simulink model "VACModel"  (Simulink 8.3)
(part 6 of 18)

      |         SW_signal = evalin('base', SW_signal);
      |         if ~isvector(SW_signal)
      |             set_param(gcb, 'signalin', '');
      |             set_param([gcb '/SignalIn'], 'VariableName', '[]');
      |             warning(['Variable ' SW_signal ' must be a vector.']);
      |             clear SW_signal;
      |             return;
      |         end
      |         SW_stime = str2num(get_param(gcb, 'stime'));
      |         if isempty(SW_stime) || SW_stime < -1 || (SW_stime < 0 && SW_stime > -1)
      |             set_param(gcb, 'stime', '-1');
      |             SW_stime = -1;
      |             warning('Sample time must be a positive double or -1 for inherited value.');
      |         end
      | 
      |         if SW_stime == 0 || SW_stime == -1
      |             SW_stime = evalin('base', 'Ts_base');
      |         end
      | 
      |         SW_start = str2num(get_param(gcb, 'start'));
      |         SW_start = SW_stime * ceil(SW_start/SW_stime);
      |         signalstruct.time = SW_start:SW_stime:(SW_stime*(length(SW_signal) - 1) + SW_start);
      |         signalstruct.signals.values = SW_signal;
      | 
      | 		if strcmp(get_param(gcb, 'afterend'), 'Cyclic repetition')
      | 			SW_end = str2double(get_param(gcr, 'StopTime'));
      | 			while signalstruct.time(end) < SW_end
      | 				signalstruct.signals.values = [signalstruct.signals.values signalstruct.signals.values];
      | 				signalstruct.time = [signalstruct.time signalstruct.time+(signalstruct.time(end)-signalstruct.time(1))];
      | 			end
      | 		end
      | 
      | 		signalstruct.signals.values = signalstruct.signals.values(:);
      | 		signalstruct.time = signalstruct.time(:);
      |         %assignin('base', 'signalstruct', signalstruct)
      |         set_param([gcb '/SignalIn'], 'VariableName', 'signalstruct');
      |     end
      | 
      |     clear SW_signal;
      | 	clear SW_start;
      |     clear SW_stime;
      | 	clear SW_end;
      | elseif ~strcmpi(get_param(gcb, 'switch_mode'), 'Custom attack') && exists_block([gcb '/SignalIn']) % delete block
      |     delete_line(gcb, 'SignalIn/1', 'Multiport Switch/3');
      |     delete_block([gcb '/SignalIn']);
      |     % replace with constant value
      |     add_block(['built-in/Constant'], [gcb '/ReplaceBlock'], 'Position', [50 400 120 430]);
      |     add_line(gcb, ['ReplaceBlock/1'], 'Multiport Switch/3', 'autorouting', 'on');
      | end
      mask TypeOptions atkMode: Attack Type Controller/atkMode
      mask Callback atkMode:
      | AM_MaskEnables = get_param(gcb, 'MaskEnables');
      | switch get_param(gcb, 'atkMode');
      |     case 'No attack'
      |         AM_MaskEnables{3} = 'off';
      |         AM_MaskEnables{4} = 'off';
      |     case 'Step attack'
      |         AM_MaskEnables{3} = 'on';
      |         AM_MaskEnables{4} = 'off';
      |     otherwise
      |         AM_MaskEnables{3} = 'on';
      |         AM_MaskEnables{4} = 'on';
      | end
      | set_param(gcb, 'MaskEnables', AM_MaskEnables);
      | 
      | clear AM_MaskEnables;
      mask Callback start:
      | SS_start = get_param(gcb, 'start');
      | if strcmp(SS_start, '') % empty
      |     set_param(gcb, 'start', '0');
      |     SS_start = 0;
      | end
      | SS_start = str2num(SS_start);
      | if isempty(SS_start)
      |     set_param(gcb, 'start', '0');
      |     SS_start = 0;
      |     warning('Parameter value must be a nimeric value.');
      | end
      | 
      | % set to the subsystem
      | set_param([gcb '/Attack Type Controller'], 'start', get_param(gcb, 'start'));
      | 
      | % get correct signal parameters
      | if strcmpi(get_param(gcb, 'switch_mode'),'custom attack')
      |     if ~exists_block([gcb '/SignalIn'])
      |         clear SS_start;
      |         return
      |     end
      |     % forward signal parameters if set
      |     SS_signal = get_param(gcb, 'signalin');
      |     if strcmp(SS_signal, '[]') || strcmp(SS_signal, '') % signal not set
      |         clear SS_signal;
      |         clear SS_start;
      |         return;
      |     else    % signal set
      |         SS_signal = evalin('base', SS_signal);
      |         SS_stime = str2num(get_param(gcb, 'stime'));
      |         if isempty(SS_stime) || SS_stime < -1 || (SS_stime < 0 && SS_stime > -1)
      |             clear SS_signal;
      |             clear SS_start;
      |             set_param(gcb, 'stime', '-1');
      |             SS_stime = -1;
      |             warning('Sample time must be a positve double or -1 for inherited value.')
      |         end
      | 
      |         if SS_stime == 0 || SS_stime == -1
      |             SS_stime = evalin('base', 'Ts_base');
      |         end
      | 
      | 
      |         signalstruct.time = SS_start:SS_stime:(SS_stime*(length(SS_signal) - 1) + SS_start);
      |         signalstruct.signals.values = SS_signal;
      | 
      | 		if strcmp(get_param(gcb, 'afterend'), 'Cyclic repetition')
      | 			SS_end = str2double(get_param(gcr, 'StopTime'));
      | 			while signalstruct.time(end) < SS_end
      | 				signalstruct.signals.values = [signalstruct.signals.values signalstruct.signals.values];
      | 				signalstruct.time = [signalstruct.time signalstruct.time+(signalstruct.time(end)-signalstruct.time(1))];
      | 			end
      | 		end
      | 
      | 		signalstruct.signals.values = signalstruct.signals.values(:);
      | 		signalstruct.time = signalstruct.time(:);
      |         %assignin('base', 'signalstruct', signalstruct)
      |         set_param([gcb '/SignalIn'], 'VariableName', 'signalstruct');
      | 		clear SS_signal;
      | 		clear SS_start;
      | 		clear SS_stime;
      | 		clear SS_end;
      |     end
      | 
      | end
      mask TypeOptions duration: Attack Type Controller/duration
      mask TypeOptions Value: Integrity attack value/Value
      mask Callback signalin:
      | if ~exists_block([gcb '/SignalIn'])
      |     return;
      | end
      | 
      | % forward signal parameters if set
      | SI_signal = get_param(gcb, 'signalin');
      | if strcmp(SI_signal, '[]') || strcmp(SI_signal, '') % signal not set
      |     set_param([gcb '/SignalIn'], 'VariableName', '[]');
      |     set_param(gcb, 'signalin', '[]');
      |     clear SI_signal;
      | else
      |     if ~exist(SI_signal)
      |         set_param(gcb, 'signalin', '[]');
      |         set_param([gcb '/SignalIn'], 'VariableName', '[]');
      |         warning('VAC:AttackController:Signal variable', ['Variable ' SI_signal ' not found.']);
      |         clear SI_signal;
      |         return;
      |     end
      | 
      |     SI_signal = evalin('base', SI_signal);
      |     if ~isvector(SI_signal)
      |         set_param(gcb, 'signalin', '[]');
      |         set_param([gcb '/SignalIn'], 'VariableName', '[]');
      |         warning('VAC:AttackController:Signal variable', ['Variable ' SI_signal ' must be a vector.']);
      |         clear SI_signal;
      |         return;
      |     end
      | 
      |     SI_stime = str2num(get_param(gcb, 'stime'));
      |     if isempty(SI_stime) || SI_stime < -1 || (SI_stime < 0 && SI_stime > -1)
      |         set_param(gcb, 'stime', '-1');
      |         SI_stime = -1;
      |         warning('VAC:AttackController:Signal variable', 'Sample time must be a positive double or -1 for inherited value.');
      |     end
      | 
      |     if SI_stime == 0 || SI_stime == -1
      |         SI_stime = evalin('base', 'Ts_base');
      |     end
      | 
      | 	SI_start = str2double(get_param(gcb, 'start'));
      | 	SI_start = SI_stime * ceil(SI_start/SI_stime);
      | 	signalstruct.time = SI_start:SI_stime:(SI_stime*(length(SI_signal) - 1) + SI_start);
      | 	signalstruct.signals.values = SI_signal;
      | 
      |     if strcmp(get_param(gcb, 'afterend'), 'Cyclic repetition')
      | 		SI_end = str2double(get_param(gcr, 'StopTime'));
      | 		while signalstruct.time(end) < SI_end
      | 			signalstruct.signals.values = [signalstruct.signals.values signalstruct.signals.values];
      | 			signalstruct.time = [signalstruct.time signalstruct.time+(signalstruct.time(end)-signalstruct.time(1))];
      | 		end
      | 	end
      | 
      | 	signalstruct.signals.values = signalstruct.signals.values(:);
      | 	signalstruct.time = signalstruct.time(:);
      |     %assignin('base', 'signalstruct', signalstruct)
      |     set_param([gcb '/SignalIn'], 'VariableName', 'signalstruct');
      | 	clear SI_stime;
      | 	clear SI_start;
      | 	clear SI_signal;
      | 	clear SI_end;
      | end
      mask Callback stime:
      | SQ_stime = get_param(gcb, 'stime');
      | if strcmp(SQ_stime, '') % empty
      |     set_param(gcb, 'stime', '-1');
      |     SQ_stime = -1;
      | end
      | SQ_stime = str2num(SQ_stime);
      | if isempty(SQ_stime)
      |     set_param(gcb, 'stime', '-1');
      |     SQ_stime = -1;
      |     warning('VAC:AttackController:Sample time','Sample time must be a positve double or -1 for inherited value.')
      | end
      | 
      | % get correct signal parameters
      | if strcmpi(get_param(gcb, 'switch_mode'),'custom attack')
      |     if ~exists_block([gcb '/SignalIn'])
      |         clear SS_start;
      |         return
      |     end
      |     % forward signal parameters if set
      |     SQ_signal = get_param(gcb, 'signalin');
      |     if strcmp(SQ_signal, '[]') || strcmp(SQ_signal, '') % signal not set
      |         clear SQ_signal;
      |         clear SQ_stime;
      |         return;
      |     else    % signal set
      |         SQ_signal = evalin('base', SQ_signal);
      |         if SQ_stime == 0 || SQ_stime == -1
      |             SQ_stime = evalin('base', 'Ts_base');
      |         end
      | 
      | 		SQ_start = str2double(get_param(gcb, 'start'));
      | 		SQ_start = SQ_stime * ceil(SQ_start/SQ_stime);
      | 		signalstruct.time = SQ_start:SQ_stime:(SQ_stime*(length(SQ_signal) - 1) + SQ_start);
      |         signalstruct.signals.values = SQ_signal;
      | 
      | 		if strcmp(get_param(gcb, 'afterend'), 'Cyclic repetition')
      | 			SQ_end = str2double(get_param(gcr, 'StopTime'));
      | 			while signalstruct.time(end) < SQ_end
      | 				signalstruct.signals.values = [signalstruct.signals.values signalstruct.signals.values];
      | 				signalstruct.time = [signalstruct.time signalstruct.time+(signalstruct.time(end)-signalstruct.time(1))];
      | 			end
      | 		end
      | 
      | 		signalstruct.signals.values = signalstruct.signals.values(:);
      | 		signalstruct.time = signalstruct.time(:);
      |         %assignin('base', 'signalstruct', signalstruct)
      |         set_param([gcb '/SignalIn'], 'VariableName', 'signalstruct');
      |     end
      | 	clear SQ_signal;
      | 	clear SQ_start;
      | 	clear SQ_stime;
      | 	clear SQ_end;
      | end
      mask TypeOptions afterend: Extrapolation | Setting to zero | Holding final value | Cyclic repetition
      mask Callback afterend:
      | if ~exists_block([gcb '/SignalIn'])
      |     return
      | end
      | 
      | % forward choosen value
      | if ~strcmp(get_param(gcb, 'afterend'), 'Cyclic repetition')
      | 	set_param([gcb '/SignalIn'], 'OutputAfterFinalValue', get_param(gcb, 'afterend'));
      | end
      | 
      | % forward signal parameters if set
      | SA_signal = get_param(gcb, 'signalin');
      | if strcmp(SA_signal, '[]') || strcmp(SA_signal, '') % signal not set
      |     set_param([gcb '/SignalIn'], 'VariableName', '[]');
      |     set_param(gcb, 'signalin', '[]');
      |     clear SA_signal;
      | else
      |     if ~exist(SA_signal)
      |         set_param(gcb, 'signalin', '[]');
      |         set_param([gcb '/SignalIn'], 'VariableName', '[]');
      |         warning('VAC:AttackController:After end', ['Variable ' SA_signal ' not found.']);
      |         clear SA_signal;
      |         return;
      |     end
      | 
      |     SA_signal = evalin('base', SA_signal);
      |     if ~isvector(SA_signal)
      |         set_param(gcb, 'signalin', '[]');
      |         set_param([gcb '/SignalIn'], 'VariableName', '[]');
      |         warning('VAC:AttackController:After end', ['Variable ' SA_signal ' must be a vector.']);
      |         clear SA_signal;
      |         return;
      |     end
      | 
      |     SA_stime = str2num(get_param(gcb, 'stime'));
      |     if isempty(SA_stime) || SA_stime < -1 || (SA_stime < 0 && SA_stime > -1)
      |         set_param(gcb, 'stime', '-1');
      |         SA_stime = -1;
      |         warning('VAC:AttackController:After end', 'Sample time must be a positive double or -1 for inherited value.');
      |     end
      | 
      |     if SA_stime == 0 || SA_stime == -1
      |         SA_stime = evalin('base', 'Ts_base');
      |     end
      | 
      | 	SA_start = str2double(get_param(gcb, 'start'));
      | 	SA_start = SA_stime * ceil(SA_start/SA_stime);
      | 	signalstruct.time = SA_start:SA_stime:(SA_stime*(length(SA_signal) - 1) + SA_start);
      | 	signalstruct.signals.values = SA_signal;
      | 
      | 	if strcmp(get_param(gcb, 'afterend'), 'Cyclic repetition')
      | 		SA_end = str2double(get_param(gcr, 'StopTime'));
      | 		while signalstruct.time(end) < SA_end
      | 			signalstruct.signals.values = [signalstruct.signals.values signalstruct.signals.values];
      | 			signalstruct.time = [signalstruct.time signalstruct.time+(signalstruct.time(end)-signalstruct.time(1))];
      | 		end
      |     end
      | 
      |     signalstruct.time = signalstruct.time(:);
      | 	signalstruct.signals.values = signalstruct.signals.values(:);
      |     %assignin('base', 'signalstruct', signalstruct)
      |     set_param([gcb '/SignalIn'], 'VariableName', 'signalstruct');
      | 
      | 	clear SA_stime;
      | 	clear SA_start;
      | 	clear SA_signal;
      | 	clear SA_end;
      | end
      mask Display:
      | disp([get_param(gcb, 'switch_mode') '\n' get_param(gcb, 'atkMode')])
      | port_label('input', 1, 'signal in')
      | port_label('output', 1, 'signal out')
  xmeas39 attack controller : Subsystem  AncestorBlock=VAlib/Attack Controller  mask(Attack controller){switch_mode=Integrity attack, atkMode=No attack, start=1, duration=1, Value=0, signalin=[], stime=-1, afterend=Holding final value}
      mask prompts: switch_mode "Attack Type:"; atkMode "Attack Mode:"; Value "Integrity Attack Value:"; signalin "Signal variable:"; stime "Sample time:"; afterend "Output after final:"
      mask help:
      | Attack controller block controls an attack on choosen variable on the specified time.
      | Attack types: DoS, Integrity and custom signal attack.
      | Modes: Step attack on specified time, Interval to specified time, Periodic and no attack.
      mask TypeOptions switch_mode: Integrity attack | DOS attack | Custom attack
      mask Callback switch_mode:
      | SM_MaskEnables = get_param(gcb, 'MaskEnables');
      | switch get_param(gcb, 'switch_mode')
      |     case 'Integrity attack'
      |         set_param([gcb,'/Switch value'], 'Value', '1');
      |         SM_MaskEnables{5} = 'on';
      |         SM_MaskEnables{6} = 'off';
      |         SM_MaskEnables{7} = 'off';
      |         SM_MaskEnables{8} = 'off';
      |     case 'DOS attack'
      |         set_param([gcb,'/Switch value'], 'Value', '3');
      |         SM_MaskEnables{5} = 'off';
      |         SM_MaskEnables{6} = 'off';
      |         SM_MaskEnables{7} = 'off';
      |         SM_MaskEnables{8} = 'off';
      |     case 'Custom attack'
      |         set_param([gcb,'/Switch value'], 'Value', '2');
      |         SM_MaskEnables{5} = 'off';
      |         SM_MaskEnables{6} = 'on';
      |         SM_MaskEnables{7} = 'on';
      |         SM_MaskEnables{8} = 'on';
      | end
      | set_param(gcb,'MaskEnables',SM_MaskEnables);
      | clear SM_MaskEnables;
      | 
      | % creat or remove block for custom attack
      | if strcmpi(get_param(gcb, 'switch_mode'), 'Custom attack') && ~exists_block([gcb '/SignalIn']) % creat block
      |     if exists_block([gcb, '/ReplaceBlock']);
      |         delete_line(gcb, 'ReplaceBlock/1', 'Multiport Switch/3');
      |         delete_block([gcb '/ReplaceBlock']);
      |     end
      | 
      |     add_block('built-in/FromWorkspace', [gcb '/SignalIn'], 'Position', [50 400 120 430]);
      |     add_line(gcb, 'SignalIn/1', 'Multiport Switch/3', 'autorouting', 'on');
      |     %set params
      |     set_param([gcb '/SignalIn'], 'SampleTime', '0');
      |     %set_param([gcb '/SignalIn'], 'VariableName', '[]');
      |     set_param([gcb '/SignalIn'], 'Interpolate', 'on');
      |     set_param([gcb '/SignalIn'], 'ZeroCross', 'off');
      |     %set_param([gcb '/' name], 'OutputAfterFinalValue', 'Setting to zero');
      |     %set_param([gcb '/' name], 'OutputAfterFinalValue', 'Cyclic repetition');
      |     %set_param([gcb '/' name], 'OutputAfterFinalValue', 'Extrapolation');
      |     %set_param([gcb '/' name], 'OutputAfterFinalValue', 'Holding final value');
      | 
      |     % forward signal parameters if set
      |     SW_signal = get_param(gcb, 'signalin');
      |     if strcmp(SW_signal, '[]') || strcmp(SW_signal, '') % signal not set
      |         set_param(gcb, 'signalin', '[]');
      |         set_param([gcb '/SignalIn'], 'VariableName', '[]');
      |         clear SW_signal;
      |         return;
      |     else    % signal set
      |         % check signal
      |         if ~exist(SW_signal)
      |             set_param(gcb, 'signalin', '[]');
      |             set_param([gcb '/SignalIn'], 'VariableName', '[]');
      |             warning(['Variable ' SW_signal ' not found.']);
      |             clear SW_signal;
      |             return;
      |         end
      |         SW_signal = evalin('base', SW_signal);
      |         if ~isvector(SW_signal)
      |             set_param(gcb, 'signalin', '');
      |             set_param([gcb '/SignalIn'], 'VariableName', '[]');
      |             warning(['Variable ' SW_signal ' must be a vector.']);
      |             clear SW_signal;
      |             return;
      |         end
      |         SW_stime = str2num(get_param(gcb, 'stime'));
      |         if isempty(SW_stime) || SW_stime < -1 || (SW_stime < 0 && SW_stime > -1)
      |             set_param(gcb, 'stime', '-1');
      |             SW_stime = -1;
      |             warning('Sample time must be a positive double or -1 for inherited value.');
      |         end
      | 
      |         if SW_stime == 0 || SW_stime == -1
      |             SW_stime = evalin('base', 'Ts_base');
      |         end
      | 
      |         SW_start = str2num(get_param(gcb, 'start'));
      |         SW_start = SW_stime * ceil(SW_start/SW_stime);
      |         signalstruct.time = SW_start:SW_stime:(SW_stime*(length(SW_signal) - 1) + SW_start);
      |         signalstruct.signals.values = SW_signal;
      | 
      | 		if strcmp(get_param(gcb, 'afterend'), 'Cyclic repetition')
      | 			SW_end = str2double(get_param(gcr, 'StopTime'));
      | 			while signalstruct.time(end) < SW_end
      | 				signalstruct.signals.values = [signalstruct.signals.values signalstruct.signals.values];
      | 				signalstruct.time = [signalstruct.time signalstruct.time+(signalstruct.time(end)-signalstruct.time(1))];
      | 			end
      | 		end
      | 
      | 		signalstruct.signals.values = signalstruct.signals.values(:);
      | 		signalstruct.time = signalstruct.time(:);
      |         %assignin('base', 'signalstruct', signalstruct)
      |         set_param([gcb '/SignalIn'], 'VariableName', 'signalstruct');
      |     end
      | 
      |     clear SW_signal;
      | 	clear SW_start;
      |     clear SW_stime;
      | 	clear SW_end;
      | elseif ~strcmpi(get_param(gcb, 'switch_mode'), 'Custom attack') && exists_block([gcb '/SignalIn']) % delete block
      |     delete_line(gcb, 'SignalIn/1', 'Multiport Switch/3');
      |     delete_block([gcb '/SignalIn']);
      |     % replace with constant value
      |     add_block(['built-in/Constant'], [gcb '/ReplaceBlock'], 'Position', [50 400 120 430]);
      |     add_line(gcb, ['ReplaceBlock/1'], 'Multiport Switch/3', 'autorouting', 'on');
      | end
      mask TypeOptions atkMode: Attack Type Controller/atkMode
      mask Callback atkMode:
      | AM_MaskEnables = get_param(gcb, 'MaskEnables');
      | switch get_param(gcb, 'atkMode');
      |     case 'No attack'
      |         AM_MaskEnables{3} = 'off';
      |         AM_MaskEnables{4} = 'off';
      |     case 'Step attack'
      |         AM_MaskEnables{3} = 'on';
      |         AM_MaskEnables{4} = 'off';
      |     otherwise
      |         AM_MaskEnables{3} = 'on';
      |         AM_MaskEnables{4} = 'on';
      | end
      | set_param(gcb, 'MaskEnables', AM_MaskEnables);
      | 
      | clear AM_MaskEnables;
      mask Callback start:
      | SS_start = get_param(gcb, 'start');
      | if strcmp(SS_start, '') % empty
      |     set_param(gcb, 'start', '0');
      |     SS_start = 0;
      | end
      | SS_start = str2num(SS_start);
      | if isempty(SS_start)
      |     set_param(gcb, 'start', '0');
      |     SS_start = 0;
      |     warning('Parameter value must be a nimeric value.');
      | end
      | 
      | % set to the subsystem
      | set_param([gcb '/Attack Type Controller'], 'start', get_param(gcb, 'start'));
      | 
      | % get correct signal parameters
      | if strcmpi(get_param(gcb, 'switch_mode'),'custom attack')
      |     if ~exists_block([gcb '/SignalIn'])
      |         clear SS_start;
      |         return
      |     end
      |     % forward signal parameters if set
      |     SS_signal = get_param(gcb, 'signalin');
      |     if strcmp(SS_signal, '[]') || strcmp(SS_signal, '') % signal not set
      |         clear SS_signal;
      |         clear SS_start;
      |         return;
      |     else    % signal set
      |         SS_signal = evalin('base', SS_signal);
      |         SS_stime = str2num(get_param(gcb, 'stime'));
      |         if isempty(SS_stime) || SS_stime < -1 || (SS_stime < 0 && SS_stime > -1)
      |             clear SS_signal;
      |             clear SS_start;
      |             set_param(gcb, 'stime', '-1');
      |             SS_stime = -1;
      |             warning('Sample time must be a positve double or -1 for inherited value.')
      |         end
      | 
      |         if SS_stime == 0 || SS_stime == -1
      |             SS_stime = evalin('base', 'Ts_base');
      |         end
      | 
      | 
      |         signalstruct.time = SS_start:SS_stime:(SS_stime*(length(SS_signal) - 1) + SS_start);
      |         signalstruct.signals.values = SS_signal;
      | 
      | 		if strcmp(get_param(gcb, 'afterend'), 'Cyclic repetition')
      | 			SS_end = str2double(get_param(gcr, 'StopTime'));
      | 			while signalstruct.time(end) < SS_end
      | 				signalstruct.signals.values = [signalstruct.signals.values signalstruct.signals.values];
      | 				signalstruct.time = [signalstruct.time signalstruct.time+(signalstruct.time(end)-signalstruct.time(1))];
      | 			end
      | 		end
      | 
      | 		signalstruct.signals.values = signalstruct.signals.values(:);
      | 		signalstruct.time = signalstruct.time(:);
      |         %assignin('base', 'signalstruct', signalstruct)
      |         set_param([gcb '/SignalIn'], 'VariableName', 'signalstruct');
      | 		clear SS_signal;
      | 		clear SS_start;
      | 		clear SS_stime;
      | 		clear SS_end;
      |     end
      | 
      | end
      mask TypeOptions duration: Attack Type Controller/duration
      mask TypeOptions Value: Integrity attack value/Value
      mask Callback signalin:
      | if ~exists_block([gcb '/SignalIn'])
      |     return;
      | end
      | 
      | % forward signal parameters if set
      | SI_signal = get_param(gcb, 'signalin');
      | if strcmp(SI_signal, '[]') || strcmp(SI_signal, '') % signal not set
      |     set_param([gcb '/SignalIn'], 'VariableName', '[]');
      |     set_param(gcb, 'signalin', '[]');
      |     clear SI_signal;
      | else
      |     if ~exist(SI_signal)
      |         set_param(gcb, 'signalin', '[]');
      |         set_param([gcb '/SignalIn'], 'VariableName', '[]');
      |         warning('VAC:AttackController:Signal variable', ['Variable ' SI_signal ' not found.']);
      |         clear SI_signal;
      |         return;
      |     end
      | 
      |     SI_signal = evalin('base', SI_signal);
      |     if ~isvector(SI_signal)
      |         set_param(gcb, 'signalin', '[]');
      |         set_param([gcb '/SignalIn'], 'VariableName', '[]');
      |         warning('VAC:AttackController:Signal variable', ['Variable ' SI_signal ' must be a vector.']);
      |         clear SI_signal;
      |         return;
      |     end
      | 
      |     SI_stime = str2num(get_param(gcb, 'stime'));
      |     if isempty(SI_stime) || SI_stime < -1 || (SI_stime < 0 && SI_stime > -1)
      |         set_param(gcb, 'stime', '-1');
      |         SI_stime = -1;
      |         warning('VAC:AttackController:Signal variable', 'Sample time must be a positive double or -1 for inherited value.');
      |     end
      | 
      |     if SI_stime == 0 || SI_stime == -1
      |         SI_stime = evalin('base', 'Ts_base');
      |     end
      | 
      | 	SI_start = str2double(get_param(gcb, 'start'));
      | 	SI_start = SI_stime * ceil(SI_start/SI_stime);
      | 	signalstruct.time = SI_start:SI_stime:(SI_stime*(length(SI_signal) - 1) + SI_start);
      | 	signalstruct.signals.values = SI_signal;
      | 
      |     if strcmp(get_param(gcb, 'afterend'), 'Cyclic repetition')
      | 		SI_end = str2double(get_param(gcr, 'StopTime'));
      | 		while signalstruct.time(end) < SI_end
      | 			signalstruct.signals.values = [signalstruct.signals.values signalstruct.signals.values];
      | 			signalstruct.time = [signalstruct.time signalstruct.time+(signalstruct.time(end)-signalstruct.time(1))];
      | 		end
      | 	end
      | 
      | 	signalstruct.signals.values = signalstruct.signals.values(:);
      | 	signalstruct.time = signalstruct.time(:);
      |     %assignin('base', 'signalstruct', signalstruct)
      |     set_param([gcb '/SignalIn'], 'VariableName', 'signalstruct');
      | 	clear SI_stime;
      | 	clear SI_start;
      | 	clear SI_signal;
      | 	clear SI_end;
      | end
      mask Callback stime:
      | SQ_stime = get_param(gcb, 'stime');
      | if strcmp(SQ_stime, '') % empty
      |     set_param(gcb, 'stime', '-1');
      |     SQ_stime = -1;
      | end
      | SQ_stime = str2num(SQ_stime);
      | if isempty(SQ_stime)
      |     set_param(gcb, 'stime', '-1');
      |     SQ_stime = -1;
      |     warning('VAC:AttackController:Sample time','Sample time must be a positve double or -1 for inherited value.')
      | end
      | 
      | % get correct signal parameters
      | if strcmpi(get_param(gcb, 'switch_mode'),'custom attack')
      |     if ~exists_block([gcb '/SignalIn'])
      |         clear SS_start;
      |         return
      |     end
      |     % forward signal parameters if set
      |     SQ_signal = get_param(gcb, 'signalin');
      |     if strcmp(SQ_signal, '[]') || strcmp(SQ_signal, '') % signal not set
      |         clear SQ_signal;
      |         clear SQ_stime;
      |         return;
      |     else    % signal set
      |         SQ_signal = evalin('base', SQ_signal);
      |         if SQ_stime == 0 || SQ_stime == -1
      |             SQ_stime = evalin('base', 'Ts_base');
      |         end
      | 
      | 		SQ_start = str2double(get_param(gcb, 'start'));
      | 		SQ_start = SQ_stime * ceil(SQ_start/SQ_stime);
      | 		signalstruct.time = SQ_start:SQ_stime:(SQ_stime*(length(SQ_signal) - 1) + SQ_start);
      |         signalstruct.signals.values = SQ_signal;
      | 
      | 		if strcmp(get_param(gcb, 'afterend'), 'Cyclic repetition')
      | 			SQ_end = str2double(get_param(gcr, 'StopTime'));
      | 			while signalstruct.time(end) < SQ_end
      | 				signalstruct.signals.values = [signalstruct.signals.values signalstruct.signals.values];
      | 				signalstruct.time = [signalstruct.time signalstruct.time+(signalstruct.time(end)-signalstruct.time(1))];
      | 			end
      | 		end
      | 
      | 		signalstruct.signals.values = signalstruct.signals.values(:);
      | 		signalstruct.time = signalstruct.time(:);
      |         %assignin('base', 'signalstruct', signalstruct)
      |         set_param([gcb '/SignalIn'], 'VariableName', 'signalstruct');
      |     end
      | 	clear SQ_signal;
      | 	clear SQ_start;
      | 	clear SQ_stime;
      | 	clear SQ_end;
      | end
      mask TypeOptions afterend: Extrapolation | Setting to zero | Holding final value | Cyclic repetition
      mask Callback afterend:
      | if ~exists_block([gcb '/SignalIn'])
      |     return
      | end
      | 
      | % forward choosen value
      | if ~strcmp(get_param(gcb, 'afterend'), 'Cyclic repetition')
      | 	set_param([gcb '/SignalIn'], 'OutputAfterFinalValue', get_param(gcb, 'afterend'));
      | end
      | 
      | % forward signal parameters if set
      | SA_signal = get_param(gcb, 'signalin');
      | if strcmp(SA_signal, '[]') || strcmp(SA_signal, '') % signal not set
      |     set_param([gcb '/SignalIn'], 'VariableName', '[]');
      |     set_param(gcb, 'signalin', '[]');
      |     clear SA_signal;
      | else
      |     if ~exist(SA_signal)
      |         set_param(gcb, 'signalin', '[]');
      |         set_param([gcb '/SignalIn'], 'VariableName', '[]');
      |         warning('VAC:AttackController:After end', ['Variable ' SA_signal ' not found.']);
      |         clear SA_signal;
      |         return;
      |     end
      | 
      |     SA_signal = evalin('base', SA_signal);
      |     if ~isvector(SA_signal)
      |         set_param(gcb, 'signalin', '[]');
      |         set_param([gcb '/SignalIn'], 'VariableName', '[]');
      |         warning('VAC:AttackController:After end', ['Variable ' SA_signal ' must be a vector.']);
      |         clear SA_signal;
      |         return;
      |     end
      | 
      |     SA_stime = str2num(get_param(gcb, 'stime'));
      |     if isempty(SA_stime) || SA_stime < -1 || (SA_stime < 0 && SA_stime > -1)
      |         set_param(gcb, 'stime', '-1');
      |         SA_stime = -1;
      |         warning('VAC:AttackController:After end', 'Sample time must be a positive double or -1 for inherited value.');
      |     end
      | 
      |     if SA_stime == 0 || SA_stime == -1
      |         SA_stime = evalin('base', 'Ts_base');
      |     end
      | 
      | 	SA_start = str2double(get_param(gcb, 'start'));
      | 	SA_start = SA_stime * ceil(SA_start/SA_stime);
      | 	signalstruct.time = SA_start:SA_stime:(SA_stime*(length(SA_signal) - 1) + SA_start);
      | 	signalstruct.signals.values = SA_signal;
      | 
      | 	if strcmp(get_param(gcb, 'afterend'), 'Cyclic repetition')
      | 		SA_end = str2double(get_param(gcr, 'StopTime'));
      | 		while signalstruct.time(end) < SA_end
      | 			signalstruct.signals.values = [signalstruct.signals.values signalstruct.signals.values];
      | 			signalstruct.time = [signalstruct.time signalstruct.time+(signalstruct.time(end)-signalstruct.time(1))];
      | 		end
      |     end
      | 
      |     signalstruct.time = signalstruct.time(:);
      | 	signalstruct.signals.values = signalstruct.signals.values(:);
      |     %assignin('base', 'signalstruct', signalstruct)
      |     set_param([gcb '/SignalIn'], 'VariableName', 'signalstruct');
      | 
      | 	clear SA_stime;
      | 	clear SA_start;
      | 	clear SA_signal;
      | 	clear SA_end;
      | end
      mask Display:
      | disp([get_param(gcb, 'switch_mode') '\n' get_param(gcb, 'atkMode')])
      | port_label('input', 1, 'signal in')
      | port_label('output', 1, 'signal out')
  xmeas4 attack controller : Subsystem  AncestorBlock=VAlib/Attack Controller  mask(Attack controller){switch_mode=Integrity attack, atkMode=No attack, start=1, duration=1, Value=0, signalin=[], stime=-1, afterend=Holding final value}
      mask prompts: switch_mode "Attack Type:"; atkMode "Attack Mode:"; Value "Integrity Attack Value:"; signalin "Signal variable:"; stime "Sample time:"; afterend "Output after final:"
      mask help:
      | Attack controller block controls an attack on choosen variable on the specified time.
      | Attack types: DoS, Integrity and custom signal attack.
      | Modes: Step attack on specified time, Interval to specified time, Periodic and no attack.
      mask TypeOptions switch_mode: Integrity attack | DOS attack | Custom attack
      mask Callback switch_mode:
      | SM_MaskEnables = get_param(gcb, 'MaskEnables');
      | switch get_param(gcb, 'switch_mode')
      |     case 'Integrity attack'
      |         set_param([gcb,'/Switch value'], 'Value', '1');
      |         SM_MaskEnables{5} = 'on';
      |         SM_MaskEnables{6} = 'off';
      |         SM_MaskEnables{7} = 'off';
      |         SM_MaskEnables{8} = 'off';
      |     case 'DOS attack'
      |         set_param([gcb,'/Switch value'], 'Value', '3');
      |         SM_MaskEnables{5} = 'off';
      |         SM_MaskEnables{6} = 'off';
      |         SM_MaskEnables{7} = 'off';
      |         SM_MaskEnables{8} = 'off';
      |     case 'Custom attack'
      |         set_param([gcb,'/Switch value'], 'Value', '2');
      |         SM_MaskEnables{5} = 'off';
      |         SM_MaskEnables{6} = 'on';
      |         SM_MaskEnables{7} = 'on';
      |         SM_MaskEnables{8} = 'on';
      | end
      | set_param(gcb,'MaskEnables',SM_MaskEnables);
      | clear SM_MaskEnables;
      | 
      | % creat or remove block for custom attack
      | if strcmpi(get_param(gcb, 'switch_mode'), 'Custom attack') && ~exists_block([gcb '/SignalIn']) % creat block
      |     if exists_block([gcb, '/ReplaceBlock']);
      |         delete_line(gcb, 'ReplaceBlock/1', 'Multiport Switch/3');
      |         delete_block([gcb '/ReplaceBlock']);
      |     end
      | 
      |     add_block('built-in/FromWorkspace', [gcb '/SignalIn'], 'Position', [50 400 120 430]);
      |     add_line(gcb, 'SignalIn/1', 'Multiport Switch/3', 'autorouting', 'on');
      |     %set params
      |     set_param([gcb '/SignalIn'], 'SampleTime', '0');
      |     %set_param([gcb '/SignalIn'], 'VariableName', '[]');
      |     set_param([gcb '/SignalIn'], 'Interpolate', 'on');
      |     set_param([gcb '/SignalIn'], 'ZeroCross', 'off');
      |     %set_param([gcb '/' name], 'OutputAfterFinalValue', 'Setting to zero');
      |     %set_param([gcb '/' name], 'OutputAfterFinalValue', 'Cyclic repetition');
      |     %set_param([gcb '/' name], 'OutputAfterFinalValue', 'Extrapolation');
      |     %set_param([gcb '/' name], 'OutputAfterFinalValue', 'Holding final value');
      | 
      |     % forward signal parameters if set
      |     SW_signal = get_param(gcb, 'signalin');
      |     if strcmp(SW_signal, '[]') || strcmp(SW_signal, '') % signal not set
      |         set_param(gcb, 'signalin', '[]');
      |         set_param([gcb '/SignalIn'], 'VariableName', '[]');
      |         clear SW_signal;
      |         return;
      |     else    % signal set
      |         % check signal
      |         if ~exist(SW_signal)
      |             set_param(gcb, 'signalin', '[]');
      |             set_param([gcb '/SignalIn'], 'VariableName', '[]');
      |             warning(['Variable ' SW_signal ' not found.']);
      |             clear SW_signal;
      |             return;
      |         end
      |         SW_signal = evalin('base', SW_signal);
      |         if ~isvector(SW_signal)
      |             set_param(gcb, 'signalin', '');
      |             set_param([gcb '/SignalIn'], 'VariableName', '[]');
      |             warning(['Variable ' SW_signal ' must be a vector.']);
      |             clear SW_signal;
      |             return;
      |         end
      |         SW_stime = str2num(get_param(gcb, 'stime'));
      |         if isempty(SW_stime) || SW_stime < -1 || (SW_stime < 0 && SW_stime > -1)
      |             set_param(gcb, 'stime', '-1');
      |             SW_stime = -1;
      |             warning('Sample time must be a positive double or -1 for inherited value.');
      |         end
      | 
      |         if SW_stime == 0 || SW_stime == -1
      |             SW_stime = evalin('base', 'Ts_base');
      |         end
      | 
      |         SW_start = str2num(get_param(gcb, 'start'));
      |         SW_start = SW_stime * ceil(SW_start/SW_stime);
      |         signalstruct.time = SW_start:SW_stime:(SW_stime*(length(SW_signal) - 1) + SW_start);
      |         signalstruct.signals.values = SW_signal;
      | 
      | 		if strcmp(get_param(gcb, 'afterend'), 'Cyclic repetition')
      | 			SW_end = str2double(get_param(gcr, 'StopTime'));
      | 			while signalstruct.time(end) < SW_end
      | 				signalstruct.signals.values = [signalstruct.signals.values signalstruct.signals.values];
      | 				signalstruct.time = [signalstruct.time signalstruct.time+(signalstruct.time(end)-signalstruct.time(1))];
      | 			end
      | 		end
      | 
      | 		signalstruct.signals.values = signalstruct.signals.values(:);
      | 		signalstruct.time = signalstruct.time(:);
      |         %assignin('base', 'signalstruct', signalstruct)
      |         set_param([gcb '/SignalIn'], 'VariableName', 'signalstruct');
      |     end
      | 
      |     clear SW_signal;
      | 	clear SW_start;
      |     clear SW_stime;
      | 	clear SW_end;
      | elseif ~strcmpi(get_param(gcb, 'switch_mode'), 'Custom attack') && exists_block([gcb '/SignalIn']) % delete block
      |     delete_line(gcb, 'SignalIn/1', 'Multiport Switch/3');
      |     delete_block([gcb '/SignalIn']);
      |     % replace with constant value
      |     add_block(['built-in/Constant'], [gcb '/ReplaceBlock'], 'Position', [50 400 120 430]);
      |     add_line(gcb, ['ReplaceBlock/1'], 'Multiport Switch/3', 'autorouting', 'on');
      | end
      mask TypeOptions atkMode: Attack Type Controller/atkMode
      mask Callback atkMode:
      | AM_MaskEnables = get_param(gcb, 'MaskEnables');
      | switch get_param(gcb, 'atkMode');
      |     case 'No attack'
      |         AM_MaskEnables{3} = 'off';
      |         AM_MaskEnables{4} = 'off';
      |     case 'Step attack'
      |         AM_MaskEnables{3} = 'on';
      |         AM_MaskEnables{4} = 'off';
      |     otherwise
      |         AM_MaskEnables{3} = 'on';
      |         AM_MaskEnables{4} = 'on';
      | end
      | set_param(gcb, 'MaskEnables', AM_MaskEnables);
      | 
      | clear AM_MaskEnables;
      mask Callback start:
      | SS_start = get_param(gcb, 'start');
      | if strcmp(SS_start, '') % empty
      |     set_param(gcb, 'start', '0');
      |     SS_start = 0;
      | end
      | SS_start = str2num(SS_start);
      | if isempty(SS_start)
      |     set_param(gcb, 'start', '0');
      |     SS_start = 0;
      |     warning('Parameter value must be a nimeric value.');
      | end
      | 
      | % set to the subsystem
      | set_param([gcb '/Attack Type Controller'], 'start', get_param(gcb, 'start'));
      | 
      | % get correct signal parameters
      | if strcmpi(get_param(gcb, 'switch_mode'),'custom attack')
      |     if ~exists_block([gcb '/SignalIn'])
      |         clear SS_start;
      |         return
      |     end
      |     % forward signal parameters if set
      |     SS_signal = get_param(gcb, 'signalin');
      |     if strcmp(SS_signal, '[]') || strcmp(SS_signal, '') % signal not set
      |         clear SS_signal;
      |         clear SS_start;
      |         return;
      |     else    % signal set
      |         SS_signal = evalin('base', SS_signal);
      |         SS_stime = str2num(get_param(gcb, 'stime'));
      |         if isempty(SS_stime) || SS_stime < -1 || (SS_stime < 0 && SS_stime > -1)
      |             clear SS_signal;
      |             clear SS_start;
      |             set_param(gcb, 'stime', '-1');
      |             SS_stime = -1;
      |             warning('Sample time must be a positve double or -1 for inherited value.')
      |         end
      | 
      |         if SS_stime == 0 || SS_stime == -1
      |             SS_stime = evalin('base', 'Ts_base');
      |         end
      | 
      | 
      |         signalstruct.time = SS_start:SS_stime:(SS_stime*(length(SS_signal) - 1) + SS_start);
      |         signalstruct.signals.values = SS_signal;
      | 
      | 		if strcmp(get_param(gcb, 'afterend'), 'Cyclic repetition')
      | 			SS_end = str2double(get_param(gcr, 'StopTime'));
      | 			while signalstruct.time(end) < SS_end
      | 				signalstruct.signals.values = [signalstruct.signals.values signalstruct.signals.values];
      | 				signalstruct.time = [signalstruct.time signalstruct.time+(signalstruct.time(end)-signalstruct.time(1))];
      | 			end
      | 		end
      | 
      | 		signalstruct.signals.values = signalstruct.signals.values(:);
      | 		signalstruct.time = signalstruct.time(:);
      |         %assignin('base', 'signalstruct', signalstruct)
      |         set_param([gcb '/SignalIn'], 'VariableName', 'signalstruct');
      | 		clear SS_signal;
      | 		clear SS_start;
      | 		clear SS_stime;
      | 		clear SS_end;
      |     end
      | 
      | end
      mask TypeOptions duration: Attack Type Controller/duration
      mask TypeOptions Value: Integrity attack value/Value
      mask Callback signalin:
      | if ~exists_block([gcb '/SignalIn'])
      |     return;
      | end
      | 
      | % forward signal parameters if set
      | SI_signal = get_param(gcb, 'signalin');
      | if strcmp(SI_signal, '[]') || strcmp(SI_signal, '') % signal not set
      |     set_param([gcb '/SignalIn'], 'VariableName', '[]');
      |     set_param(gcb, 'signalin', '[]');
      |     clear SI_signal;
      | else
      |     if ~exist(SI_signal)
      |         set_param(gcb, 'signalin', '[]');
      |         set_param([gcb '/SignalIn'], 'VariableName', '[]');
      |         warning('VAC:AttackController:Signal variable', ['Variable ' SI_signal ' not found.']);
      |         clear SI_signal;
      |         return;
      |     end
      | 
      |     SI_signal = evalin('base', SI_signal);
      |     if ~isvector(SI_signal)
      |         set_param(gcb, 'signalin', '[]');
      |         set_param([gcb '/SignalIn'], 'VariableName', '[]');
      |         warning('VAC:AttackController:Signal variable', ['Variable ' SI_signal ' must be a vector.']);
      |         clear SI_signal;
      |         return;
      |     end
      | 
      |     SI_stime = str2num(get_param(gcb, 'stime'));
      |     if isempty(SI_stime) || SI_stime < -1 || (SI_stime < 0 && SI_stime > -1)
      |         set_param(gcb, 'stime', '-1');
      |         SI_stime = -1;
      |         warning('VAC:AttackController:Signal variable', 'Sample time must be a positive double or -1 for inherited value.');
      |     end
      | 
      |     if SI_stime == 0 || SI_stime == -1
      |         SI_stime = evalin('base', 'Ts_base');
      |     end
      | 
      | 	SI_start = str2double(get_param(gcb, 'start'));
      | 	SI_start = SI_stime * ceil(SI_start/SI_stime);
      | 	signalstruct.time = SI_start:SI_stime:(SI_stime*(length(SI_signal) - 1) + SI_start);
      | 	signalstruct.signals.values = SI_signal;
      | 
      |     if strcmp(get_param(gcb, 'afterend'), 'Cyclic repetition')
      | 		SI_end = str2double(get_param(gcr, 'StopTime'));
      | 		while signalstruct.time(end) < SI_end
      | 			signalstruct.signals.values = [signalstruct.signals.values signalstruct.signals.values];
      | 			signalstruct.time = [signalstruct.time signalstruct.time+(signalstruct.time(end)-signalstruct.time(1))];
      | 		end
      | 	end
      | 
      | 	signalstruct.signals.values = signalstruct.signals.values(:);
      | 	signalstruct.time = signalstruct.time(:);
      |     %assignin('base', 'signalstruct', signalstruct)
      |     set_param([gcb '/SignalIn'], 'VariableName', 'signalstruct');
      | 	clear SI_stime;
      | 	clear SI_start;
      | 	clear SI_signal;
      | 	clear SI_end;
      | end
      mask Callback stime:
      | SQ_stime = get_param(gcb, 'stime');
      | if strcmp(SQ_stime, '') % empty
      |     set_param(gcb, 'stime', '-1');
      |     SQ_stime = -1;
      | end
      | SQ_stime = str2num(SQ_stime);
      | if isempty(SQ_stime)
      |     set_param(gcb, 'stime', '-1');
      |     SQ_stime = -1;
      |     warning('VAC:AttackController:Sample time','Sample time must be a positve double or -1 for inherited value.')
      | end
      | 
      | % get correct signal parameters
      | if strcmpi(get_param(gcb, 'switch_mode'),'custom attack')
      |     if ~exists_block([gcb '/SignalIn'])
      |         clear SS_start;
      |         return
      |     end
      |     % forward signal parameters if set
      |     SQ_signal = get_param(gcb, 'signalin');
      |     if strcmp(SQ_signal, '[]') || strcmp(SQ_signal, '') % signal not set
      |         clear SQ_signal;
      |         clear SQ_stime;
      |         return;
      |     else    % signal set
      |         SQ_signal = evalin('base', SQ_signal);
      |         if SQ_stime == 0 || SQ_stime == -1
      |             SQ_stime = evalin('base', 'Ts_base');
      |         end
      | 
      | 		SQ_start = str2double(get_param(gcb, 'start'));
      | 		SQ_start = SQ_stime * ceil(SQ_start/SQ_stime);
      | 		signalstruct.time = SQ_start:SQ_stime:(SQ_stime*(length(SQ_signal) - 1) + SQ_start);
      |         signalstruct.signals.values = SQ_signal;
      | 
      | 		if strcmp(get_param(gcb, 'afterend'), 'Cyclic repetition')
      | 			SQ_end = str2double(get_param(gcr, 'StopTime'));
      | 			while signalstruct.time(end) < SQ_end
      | 				signalstruct.signals.values = [signalstruct.signals.values signalstruct.signals.values];
      | 				signalstruct.time = [signalstruct.time signalstruct.time+(signalstruct.time(end)-signalstruct.time(1))];
      | 			end
      | 		end
      | 
      | 		signalstruct.signals.values = signalstruct.signals.values(:);
      | 		signalstruct.time = signalstruct.time(:);
      |         %assignin('base', 'signalstruct', signalstruct)
      |         set_param([gcb '/SignalIn'], 'VariableName', 'signalstruct');
      |     end
      | 	clear SQ_signal;
      | 	clear SQ_start;
      | 	clear SQ_stime;
      | 	clear SQ_end;
      | end
      mask TypeOptions afterend: Extrapolation | Setting to zero | Holding final value | Cyclic repetition
      mask Callback afterend:
      | if ~exists_block([gcb '/SignalIn'])
      |     return
      | end
      | 
      | % forward choosen value
      | if ~strcmp(get_param(gcb, 'afterend'), 'Cyclic repetition')
      | 	set_param([gcb '/SignalIn'], 'OutputAfterFinalValue', get_param(gcb, 'afterend'));
      | end
      | 
      | % forward signal parameters if set
      | SA_signal = get_param(gcb, 'signalin');
      | if strcmp(SA_signal, '[]') || strcmp(SA_signal, '') % signal not set
      |     set_param([gcb '/SignalIn'], 'VariableName', '[]');
      |     set_param(gcb, 'signalin', '[]');
      |     clear SA_signal;
      | else
      |     if ~exist(SA_signal)
      |         set_param(gcb, 'signalin', '[]');
      |         set_param([gcb '/SignalIn'], 'VariableName', '[]');
      |         warning('VAC:AttackController:After end', ['Variable ' SA_signal ' not found.']);
      |         clear SA_signal;
      |         return;
      |     end
      | 
      |     SA_signal = evalin('base', SA_signal);
      |     if ~isvector(SA_signal)
      |         set_param(gcb, 'signalin', '[]');
      |         set_param([gcb '/SignalIn'], 'VariableName', '[]');
      |         warning('VAC:AttackController:After end', ['Variable ' SA_signal ' must be a vector.']);
      |         clear SA_signal;
      |         return;
      |     end
      | 
      |     SA_stime = str2num(get_param(gcb, 'stime'));
      |     if isempty(SA_stime) || SA_stime < -1 || (SA_stime < 0 && SA_stime > -1)
      |         set_param(gcb, 'stime', '-1');
      |         SA_stime = -1;
      |         warning('VAC:AttackController:After end', 'Sample time must be a positive double or -1 for inherited value.');
      |     end
      | 
      |     if SA_stime == 0 || SA_stime == -1
      |         SA_stime = evalin('base', 'Ts_base');
      |     end
      | 
      | 	SA_start = str2double(get_param(gcb, 'start'));
      | 	SA_start = SA_stime * ceil(SA_start/SA_stime);
      | 	signalstruct.time = SA_start:SA_stime:(SA_stime*(length(SA_signal) - 1) + SA_start);
      | 	signalstruct.signals.values = SA_signal;
      | 
      | 	if strcmp(get_param(gcb, 'afterend'), 'Cyclic repetition')
      | 		SA_end = str2double(get_param(gcr, 'StopTime'));
      | 		while signalstruct.time(end) < SA_end
      | 			signalstruct.signals.values = [signalstruct.signals.values signalstruct.signals.values];
      | 			signalstruct.time = [signalstruct.time signalstruct.time+(signalstruct.time(end)-signalstruct.time(1))];
      | 		end
      |     end
      | 
      |     signalstruct.time = signalstruct.time(:);
      | 	signalstruct.signals.values = signalstruct.signals.values(:);
      |     %assignin('base', 'signalstruct', signalstruct)
      |     set_param([gcb '/SignalIn'], 'VariableName', 'signalstruct');
      | 
      | 	clear SA_stime;
      | 	clear SA_start;
      | 	clear SA_signal;
      | 	clear SA_end;
      | end
      mask Display:
      | disp([get_param(gcb, 'switch_mode') '\n' get_param(gcb, 'atkMode')])
      | port_label('input', 1, 'signal in')
      | port_label('output', 1, 'signal out')
  xmeas40 attack controller : Subsystem  AncestorBlock=VAlib/Attack Controller  mask(Attack controller){switch_mode=Integrity attack, atkMode=No attack, start=1, duration=1, Value=0, signalin=[], stime=-1, afterend=Holding final value}
      mask prompts: switch_mode "Attack Type:"; atkMode "Attack Mode:"; Value "Integrity Attack Value:"; signalin "Signal variable:"; stime "Sample time:"; afterend "Output after final:"
      mask help:
      | Attack controller block controls an attack on choosen variable on the specified time.
      | Attack types: DoS, Integrity and custom signal attack.
      | Modes: Step attack on specified time, Interval to specified time, Periodic and no attack.
      mask TypeOptions switch_mode: Integrity attack | DOS attack | Custom attack
      mask Callback switch_mode:
      | SM_MaskEnables = get_param(gcb, 'MaskEnables');
      | switch get_param(gcb, 'switch_mode')
      |     case 'Integrity attack'
      |         set_param([gcb,'/Switch value'], 'Value', '1');
      |         SM_MaskEnables{5} = 'on';
      |         SM_MaskEnables{6} = 'off';
      |         SM_MaskEnables{7} = 'off';
      |         SM_MaskEnables{8} = 'off';
      |     case 'DOS attack'
      |         set_param([gcb,'/Switch value'], 'Value', '3');
      |         SM_MaskEnables{5} = 'off';
      |         SM_MaskEnables{6} = 'off';
      |         SM_MaskEnables{7} = 'off';
      |         SM_MaskEnables{8} = 'off';
      |     case 'Custom attack'
      |         set_param([gcb,'/Switch value'], 'Value', '2');
      |         SM_MaskEnables{5} = 'off';
      |         SM_MaskEnables{6} = 'on';
      |         SM_MaskEnables{7} = 'on';
      |         SM_MaskEnables{8} = 'on';
      | end
      | set_param(gcb,'MaskEnables',SM_MaskEnables);
      | clear SM_MaskEnables;
      | 
      | % creat or remove block for custom attack
      | if strcmpi(get_param(gcb, 'switch_mode'), 'Custom attack') && ~exists_block([gcb '/SignalIn']) % creat block
      |     if exists_block([gcb, '/ReplaceBlock']);
      |         delete_line(gcb, 'ReplaceBlock/1', 'Multiport Switch/3');
      |         delete_block([gcb '/ReplaceBlock']);
      |     end
      | 
      |     add_block('built-in/FromWorkspace', [gcb '/SignalIn'], 'Position', [50 400 120 430]);
      |     add_line(gcb, 'SignalIn/1', 'Multiport Switch/3', 'autorouting', 'on');
      |     %set params
      |     set_param([gcb '/SignalIn'], 'SampleTime', '0');
      |     %set_param([gcb '/SignalIn'], 'VariableName', '[]');
      |     set_param([gcb '/SignalIn'], 'Interpolate', 'on');
      |     set_param([gcb '/SignalIn'], 'ZeroCross', 'off');
      |     %set_param([gcb '/' name], 'OutputAfterFinalValue', 'Setting to zero');
      |     %set_param([gcb '/' name], 'OutputAfterFinalValue', 'Cyclic repetition');
      |     %set_param([gcb '/' name], 'OutputAfterFinalValue', 'Extrapolation');
      |     %set_param([gcb '/' name], 'OutputAfterFinalValue', 'Holding final value');
      | 
      |     % forward signal parameters if set
      |     SW_signal = get_param(gcb, 'signalin');
      |     if strcmp(SW_signal, '[]') || strcmp(SW_signal, '') % signal not set
      |         set_param(gcb, 'signalin', '[]');
      |         set_param([gcb '/SignalIn'], 'VariableName', '[]');
      |         clear SW_signal;
      |         return;
      |     else    % signal set
      |         % check signal
      |         if ~exist(SW_signal)
      |             set_param(gcb, 'signalin', '[]');
      |             set_param([gcb '/SignalIn'], 'VariableName', '[]');
      |             warning(['Variable ' SW_signal ' not found.']);
      |             clear SW_signal;
      |             return;
      |         end
      |         SW_signal = evalin('base', SW_signal);
      |         if ~isvector(SW_signal)
      |             set_param(gcb, 'signalin', '');
      |             set_param([gcb '/SignalIn'], 'VariableName', '[]');
      |             warning(['Variable ' SW_signal ' must be a vector.']);
      |             clear SW_signal;
      |             return;
      |         end
      |         SW_stime = str2num(get_param(gcb, 'stime'));
      |         if isempty(SW_stime) || SW_stime < -1 || (SW_stime < 0 && SW_stime > -1)
      |             set_param(gcb, 'stime', '-1');
      |             SW_stime = -1;
      |             warning('Sample time must be a positive double or -1 for inherited value.');
      |         end
      | 
      |         if SW_stime == 0 || SW_stime == -1
      |             SW_stime = evalin('base', 'Ts_base');
      |         end
      | 
      |         SW_start = str2num(get_param(gcb, 'start'));
      |         SW_start = SW_stime * ceil(SW_start/SW_stime);
      |         signalstruct.time = SW_start:SW_stime:(SW_stime*(length(SW_signal) - 1) + SW_start);
      |         signalstruct.signals.values = SW_signal;
      | 
      | 		if strcmp(get_param(gcb, 'afterend'), 'Cyclic repetition')
      | 			SW_end = str2double(get_param(gcr, 'StopTime'));
      | 			while signalstruct.time(end) < SW_end
      | 				signalstruct.signals.values = [signalstruct.signals.values signalstruct.signals.values];
      | 				signalstruct.time = [signalstruct.time signalstruct.time+(signalstruct.time(end)-signalstruct.time(1))];
      | 			end
      | 		end
      | 
      | 		signalstruct.signals.values = signalstruct.signals.values(:);
      | 		signalstruct.time = signalstruct.time(:);
      |         %assignin('base', 'signalstruct', signalstruct)
      |         set_param([gcb '/SignalIn'], 'VariableName', 'signalstruct');
      |     end
      | 
      |     clear SW_signal;
      | 	clear SW_start;
      |     clear SW_stime;
      | 	clear SW_end;
      | elseif ~strcmpi(get_param(gcb, 'switch_mode'), 'Custom attack') && exists_block([gcb '/SignalIn']) % delete block
      |     delete_line(gcb, 'SignalIn/1', 'Multiport Switch/3');
      |     delete_block([gcb '/SignalIn']);
      |     % replace with constant value
      |     add_block(['built-in/Constant'], [gcb '/ReplaceBlock'], 'Position', [50 400 120 430]);
      |     add_line(gcb, ['ReplaceBlock/1'], 'Multiport Switch/3', 'autorouting', 'on');
      | end
      mask TypeOptions atkMode: Attack Type Controller/atkMode
      mask Callback atkMode:
      | AM_MaskEnables = get_param(gcb, 'MaskEnables');
      | switch get_param(gcb, 'atkMode');
      |     case 'No attack'
      |         AM_MaskEnables{3} = 'off';
      |         AM_MaskEnables{4} = 'off';
      |     case 'Step attack'
      |         AM_MaskEnables{3} = 'on';
      |         AM_MaskEnables{4} = 'off';
      |     otherwise
      |         AM_MaskEnables{3} = 'on';
      |         AM_MaskEnables{4} = 'on';
      | end
      | set_param(gcb, 'MaskEnables', AM_MaskEnables);
      | 
      | clear AM_MaskEnables;
      mask Callback start:
      | SS_start = get_param(gcb, 'start');
      | if strcmp(SS_start, '') % empty
      |     set_param(gcb, 'start', '0');
      |     SS_start = 0;
      | end
      | SS_start = str2num(SS_start);
      | if isempty(SS_start)
      |     set_param(gcb, 'start', '0');
      |     SS_start = 0;
      |     warning('Parameter value must be a nimeric value.');
      | end
      | 
      | % set to the subsystem
      | set_param([gcb '/Attack Type Controller'], 'start', get_param(gcb, 'start'));
      | 
      | % get correct signal parameters
      | if strcmpi(get_param(gcb, 'switch_mode'),'custom attack')
      |     if ~exists_block([gcb '/SignalIn'])
      |         clear SS_start;
      |         return
      |     end
      |     % forward signal parameters if set
      |     SS_signal = get_param(gcb, 'signalin');
      |     if strcmp(SS_signal, '[]') || strcmp(SS_signal, '') % signal not set
      |         clear SS_signal;
      |         clear SS_start;
      |         return;
      |     else    % signal set
      |         SS_signal = evalin('base', SS_signal);
      |         SS_stime = str2num(get_param(gcb, 'stime'));
      |         if isempty(SS_stime) || SS_stime < -1 || (SS_stime < 0 && SS_stime > -1)
      |             clear SS_signal;
      |             clear SS_start;
      |             set_param(gcb, 'stime', '-1');
      |             SS_stime = -1;
      |             warning('Sample time must be a positve double or -1 for inherited value.')
      |         end
      | 
      |         if SS_stime == 0 || SS_stime == -1
      |             SS_stime = evalin('base', 'Ts_base');
      |         end
      | 
      | 
      |         signalstruct.time = SS_start:SS_stime:(SS_stime*(length(SS_signal) - 1) + SS_start);
      |         signalstruct.signals.values = SS_signal;
      | 
      | 		if strcmp(get_param(gcb, 'afterend'), 'Cyclic repetition')
      | 			SS_end = str2double(get_param(gcr, 'StopTime'));
      | 			while signalstruct.time(end) < SS_end
      | 				signalstruct.signals.values = [signalstruct.signals.values signalstruct.signals.values];
      | 				signalstruct.time = [signalstruct.time signalstruct.time+(signalstruct.time(end)-signalstruct.time(1))];
      | 			end
      | 		end
      | 
      | 		signalstruct.signals.values = signalstruct.signals.values(:);
      | 		signalstruct.time = signalstruct.time(:);
      |         %assignin('base', 'signalstruct', signalstruct)
      |         set_param([gcb '/SignalIn'], 'VariableName', 'signalstruct');
      | 		clear SS_signal;
      | 		clear SS_start;
      | 		clear SS_stime;
      | 		clear SS_end;
      |     end
      | 
      | end
      mask TypeOptions duration: Attack Type Controller/duration
      mask TypeOptions Value: Integrity attack value/Value
      mask Callback signalin:
      | if ~exists_block([gcb '/SignalIn'])
      |     return;
      | end
      | 
      | % forward signal parameters if set
      | SI_signal = get_param(gcb, 'signalin');
      | if strcmp(SI_signal, '[]') || strcmp(SI_signal, '') % signal not set
      |     set_param([gcb '/SignalIn'], 'VariableName', '[]');
      |     set_param(gcb, 'signalin', '[]');
      |     clear SI_signal;
      | else
      |     if ~exist(SI_signal)
      |         set_param(gcb, 'signalin', '[]');
      |         set_param([gcb '/SignalIn'], 'VariableName', '[]');
      |         warning('VAC:AttackController:Signal variable', ['Variable ' SI_signal ' not found.']);
      |         clear SI_signal;
      |         return;
      |     end
      | 
      |     SI_signal = evalin('base', SI_signal);
      |     if ~isvector(SI_signal)
      |         set_param(gcb, 'signalin', '[]');
      |         set_param([gcb '/SignalIn'], 'VariableName', '[]');
      |         warning('VAC:AttackController:Signal variable', ['Variable ' SI_signal ' must be a vector.']);
      |         clear SI_signal;
      |         return;
      |     end
      | 
      |     SI_stime = str2num(get_param(gcb, 'stime'));
      |     if isempty(SI_stime) || SI_stime < -1 || (SI_stime < 0 && SI_stime > -1)
      |         set_param(gcb, 'stime', '-1');
      |         SI_stime = -1;
      |         warning('VAC:AttackController:Signal variable', 'Sample time must be a positive double or -1 for inherited value.');
      |     end
      | 
      |     if SI_stime == 0 || SI_stime == -1
      |         SI_stime = evalin('base', 'Ts_base');
      |     end
      | 
      | 	SI_start = str2double(get_param(gcb, 'start'));
      | 	SI_start = SI_stime * ceil(SI_start/SI_stime);
      | 	signalstruct.time = SI_start:SI_stime:(SI_stime*(length(SI_signal) - 1) + SI_start);
      | 	signalstruct.signals.values = SI_signal;
      | 
      |     if strcmp(get_param(gcb, 'afterend'), 'Cyclic repetition')
      | 		SI_end = str2double(get_param(gcr, 'StopTime'));
      | 		while signalstruct.time(end) < SI_end
      | 			signalstruct.signals.values = [signalstruct.signals.values signalstruct.signals.values];
      | 			signalstruct.time = [signalstruct.time signalstruct.time+(signalstruct.time(end)-signalstruct.time(1))];
      | 		end
      | 	end
      | 
      | 	signalstruct.signals.values = signalstruct.signals.values(:);
      | 	signalstruct.time = signalstruct.time(:);
      |     %assignin('base', 'signalstruct', signalstruct)
      |     set_param([gcb '/SignalIn'], 'VariableName', 'signalstruct');
      | 	clear SI_stime;
      | 	clear SI_start;
      | 	clear SI_signal;
      | 	clear SI_end;
      | end
      mask Callback stime:
      | SQ_stime = get_param(gcb, 'stime');
      | if strcmp(SQ_stime, '') % empty
      |     set_param(gcb, 'stime', '-1');
      |     SQ_stime = -1;
      | end
      | SQ_stime = str2num(SQ_stime);
      | if isempty(SQ_stime)
      |     set_param(gcb, 'stime', '-1');
      |     SQ_stime = -1;
      |     warning('VAC:AttackController:Sample time','Sample time must be a positve double or -1 for inherited value.')
      | end
      | 
      | % get correct signal parameters
      | if strcmpi(get_param(gcb, 'switch_mode'),'custom attack')
      |     if ~exists_block([gcb '/SignalIn'])
      |         clear SS_start;
      |         return
      |     end
      |     % forward signal parameters if set
      |     SQ_signal = get_param(gcb, 'signalin');
      |     if strcmp(SQ_signal, '[]') || strcmp(SQ_signal, '') % signal not set
      |         clear SQ_signal;
      |         clear SQ_stime;
      |         return;
      |     else    % signal set
      |         SQ_signal = evalin('base', SQ_signal);
      |         if SQ_stime == 0 || SQ_stime == -1
      |             SQ_stime = evalin('base', 'Ts_base');
      |         end
      | 
      | 		SQ_start = str2double(get_param(gcb, 'start'));
      | 		SQ_start = SQ_stime * ceil(SQ_start/SQ_stime);
      | 		signalstruct.time = SQ_start:SQ_stime:(SQ_stime*(length(SQ_signal) - 1) + SQ_start);
      |         signalstruct.signals.values = SQ_signal;
      | 
      | 		if strcmp(get_param(gcb, 'afterend'), 'Cyclic repetition')
      | 			SQ_end = str2double(get_param(gcr, 'StopTime'));
      | 			while signalstruct.time(end) < SQ_end
      | 				signalstruct.signals.values = [signalstruct.signals.values signalstruct.signals.values];
      | 				signalstruct.time = [signalstruct.time signalstruct.time+(signalstruct.time(end)-signalstruct.time(1))];
      | 			end
      | 		end
      | 
      | 		signalstruct.signals.values = signalstruct.signals.values(:);
      | 		signalstruct.time = signalstruct.time(:);
      |         %assignin('base', 'signalstruct', signalstruct)
      |         set_param([gcb '/SignalIn'], 'VariableName', 'signalstruct');
      |     end
      | 	clear SQ_signal;
      | 	clear SQ_start;
      | 	clear SQ_stime;
      | 	clear SQ_end;
      | end
      mask TypeOptions afterend: Extrapolation | Setting to zero | Holding final value | Cyclic repetition
      mask Callback afterend:
      | if ~exists_block([gcb '/SignalIn'])
      |     return
      | end
      | 
      | % forward choosen value
      | if ~strcmp(get_param(gcb, 'afterend'), 'Cyclic repetition')
      | 	set_param([gcb '/SignalIn'], 'OutputAfterFinalValue', get_param(gcb, 'afterend'));
      | end
      | 
      | % forward signal parameters if set
      | SA_signal = get_param(gcb, 'signalin');
      | if strcmp(SA_signal, '[]') || strcmp(SA_signal, '') % signal not set
      |     set_param([gcb '/SignalIn'], 'VariableName', '[]');
      |     set_param(gcb, 'signalin', '[]');
      |     clear SA_signal;
      | else
      |     if ~exist(SA_signal)
      |         set_param(gcb, 'signalin', '[]');
      |         set_param([gcb '/SignalIn'], 'VariableName', '[]');
      |         warning('VAC:AttackController:After end', ['Variable ' SA_signal ' not found.']);
      |         clear SA_signal;
      |         return;
      |     end
      | 
      |     SA_signal = evalin('base', SA_signal);
      |     if ~isvector(SA_signal)
      |         set_param(gcb, 'signalin', '[]');
      |         set_param([gcb '/SignalIn'], 'VariableName', '[]');
      |         warning('VAC:AttackController:After end', ['Variable ' SA_signal ' must be a vector.']);
      |         clear SA_signal;
      |         return;
      |     end
      | 
      |     SA_stime = str2num(get_param(gcb, 'stime'));
      |     if isempty(SA_stime) || SA_stime < -1 || (SA_stime < 0 && SA_stime > -1)
      |         set_param(gcb, 'stime', '-1');
      |         SA_stime = -1;
      |         warning('VAC:AttackController:After end', 'Sample time must be a positive double or -1 for inherited value.');
      |     end
      | 
      |     if SA_stime == 0 || SA_stime == -1
      |         SA_stime = evalin('base', 'Ts_base');
      |     end
      | 
      | 	SA_start = str2double(get_param(gcb, 'start'));
      | 	SA_start = SA_stime * ceil(SA_start/SA_stime);
      | 	signalstruct.time = SA_start:SA_stime:(SA_stime*(length(SA_signal) - 1) + SA_start);
      | 	signalstruct.signals.values = SA_signal;
      | 
      | 	if strcmp(get_param(gcb, 'afterend'), 'Cyclic repetition')
      | 		SA_end = str2double(get_param(gcr, 'StopTime'));
      | 		while signalstruct.time(end) < SA_end
      | 			signalstruct.signals.values = [signalstruct.signals.values signalstruct.signals.values];
      | 			signalstruct.time = [signalstruct.time signalstruct.time+(signalstruct.time(end)-signalstruct.time(1))];
      | 		end
      |     end
      | 
      |     signalstruct.time = signalstruct.time(:);
      | 	signalstruct.signals.values = signalstruct.signals.values(:);
      |     %assignin('base', 'signalstruct', signalstruct)
      |     set_param([gcb '/SignalIn'], 'VariableName', 'signalstruct');
      | 
      | 	clear SA_stime;
      | 	clear SA_start;
      | 	clear SA_signal;
      | 	clear SA_end;
      | end
      mask Display:
      | disp([get_param(gcb, 'switch_mode') '\n' get_param(gcb, 'atkMode')])
      | port_label('input', 1, 'signal in')
      | port_label('output', 1, 'signal out')
  xmeas41 attack controller : Subsystem  AncestorBlock=VAlib/Attack Controller  mask(Attack controller){switch_mode=Integrity attack, atkMode=No attack, start=1, duration=1, Value=0, signalin=[], stime=-1, afterend=Holding final value}
      mask prompts: switch_mode "Attack Type:"; atkMode "Attack Mode:"; Value "Integrity Attack Value:"; signalin "Signal variable:"; stime "Sample time:"; afterend "Output after final:"
      mask help:
      | Attack controller block controls an attack on choosen variable on the specified time.
      | Attack types: DoS, Integrity and custom signal attack.
      | Modes: Step attack on specified time, Interval to specified time, Periodic and no attack.
      mask TypeOptions switch_mode: Integrity attack | DOS attack | Custom attack
      mask Callback switch_mode:
      | SM_MaskEnables = get_param(gcb, 'MaskEnables');
      | switch get_param(gcb, 'switch_mode')
      |     case 'Integrity attack'
      |         set_param([gcb,'/Switch value'], 'Value', '1');
      |         SM_MaskEnables{5} = 'on';
      |         SM_MaskEnables{6} = 'off';
      |         SM_MaskEnables{7} = 'off';
      |         SM_MaskEnables{8} = 'off';
      |     case 'DOS attack'
      |         set_param([gcb,'/Switch value'], 'Value', '3');
      |         SM_MaskEnables{5} = 'off';
      |         SM_MaskEnables{6} = 'off';
      |         SM_MaskEnables{7} = 'off';
      |         SM_MaskEnables{8} = 'off';
      |     case 'Custom attack'
      |         set_param([gcb,'/Switch value'], 'Value', '2');
      |         SM_MaskEnables{5} = 'off';
      |         SM_MaskEnables{6} = 'on';
      |         SM_MaskEnables{7} = 'on';
      |         SM_MaskEnables{8} = 'on';
      | end
      | set_param(gcb,'MaskEnables',SM_MaskEnables);
      | clear SM_MaskEnables;
      | 
      | % creat or remove block for custom attack
      | if strcmpi(get_param(gcb, 'switch_mode'), 'Custom attack') && ~exists_block([gcb '/SignalIn']) % creat block
      |     if exists_block([gcb, '/ReplaceBlock']);
      |         delete_line(gcb, 'ReplaceBlock/1', 'Multiport Switch/3');
      |         delete_block([gcb '/ReplaceBlock']);
      |     end
      | 
      |     add_block('built-in/FromWorkspace', [gcb '/SignalIn'], 'Position', [50 400 120 430]);
      |     add_line(gcb, 'SignalIn/1', 'Multiport Switch/3', 'autorouting', 'on');
      |     %set params
      |     set_param([gcb '/SignalIn'], 'SampleTime', '0');
      |     %set_param([gcb '/SignalIn'], 'VariableName', '[]');
      |     set_param([gcb '/SignalIn'], 'Interpolate', 'on');
      |     set_param([gcb '/SignalIn'], 'ZeroCross', 'off');
      |     %set_param([gcb '/' name], 'OutputAfterFinalValue', 'Setting to zero');
      |     %set_param([gcb '/' name], 'OutputAfterFinalValue', 'Cyclic repetition');
      |     %set_param([gcb '/' name], 'OutputAfterFinalValue', 'Extrapolation');
      |     %set_param([gcb '/' name], 'OutputAfterFinalValue', 'Holding final value');
      | 
      |     % forward signal parameters if set
      |     SW_signal = get_param(gcb, 'signalin');
      |     if strcmp(SW_signal, '[]') || strcmp(SW_signal, '') % signal not set
      |         set_param(gcb, 'signalin', '[]');
      |         set_param([gcb '/SignalIn'], 'VariableName', '[]');
      |         clear SW_signal;
      |         return;
      |     else    % signal set
      |         % check signal
      |         if ~exist(SW_signal)
      |             set_param(gcb, 'signalin', '[]');
      |             set_param([gcb '/SignalIn'], 'VariableName', '[]');
      |             warning(['Variable ' SW_signal ' not found.']);
      |             clear SW_signal;
      |             return;
      |         end
      |         SW_signal = evalin('base', SW_signal);
      |         if ~isvector(SW_signal)
      |             set_param(gcb, 'signalin', '');
      |             set_param([gcb '/SignalIn'], 'VariableName', '[]');
      |             warning(['Variable ' SW_signal ' must be a vector.']);
      |             clear SW_signal;
      |             return;
      |         end
      |         SW_stime = str2num(get_param(gcb, 'stime'));
      |         if isempty(SW_stime) || SW_stime < -1 || (SW_stime < 0 && SW_stime > -1)
      |             set_param(gcb, 'stime', '-1');
      |             SW_stime = -1;
      |             warning('Sample time must be a positive double or -1 for inherited value.');
      |         end
      | 
      |         if SW_stime == 0 || SW_stime == -1
      |             SW_stime = evalin('base', 'Ts_base');
      |         end
      | 
      |         SW_start = str2num(get_param(gcb, 'start'));
      |         SW_start = SW_stime * ceil(SW_start/SW_stime);
      |         signalstruct.time = SW_start:SW_stime:(SW_stime*(length(SW_signal) - 1) + SW_start);
      |         signalstruct.signals.values = SW_signal;
      | 
      | 		if strcmp(get_param(gcb, 'afterend'), 'Cyclic repetition')
      | 			SW_end = str2double(get_param(gcr, 'StopTime'));
      | 			while signalstruct.time(end) < SW_end
      | 				signalstruct.signals.values = [signalstruct.signals.values signalstruct.signals.values];
      | 				signalstruct.time = [signalstruct.time signalstruct.time+(signalstruct.time(end)-signalstruct.time(1))];
      | 			end
      | 		end
      | 
      | 		signalstruct.signals.values = signalstruct.signals.values(:);
      | 		signalstruct.time = signalstruct.time(:);
      |         %assignin('base', 'signalstruct', signalstruct)
      |         set_param([gcb '/SignalIn'], 'VariableName', 'signalstruct');
      |     end
      | 
      |     clear SW_signal;
      | 	clear SW_start;
      |     clear SW_stime;
      | 	clear SW_end;
      | elseif ~strcmpi(get_param(gcb, 'switch_mode'), 'Custom attack') && exists_block([gcb '/SignalIn']) % delete block
      |     delete_line(gcb, 'SignalIn/1', 'Multiport Switch/3');
      |     delete_block([gcb '/SignalIn']);
      |     % replace with constant value
      |     add_block(['built-in/Constant'], [gcb '/ReplaceBlock'], 'Position', [50 400 120 430]);
      |     add_line(gcb, ['ReplaceBlock/1'], 'Multiport Switch/3', 'autorouting', 'on');
      | end
      mask TypeOptions atkMode: Attack Type Controller/atkMode
      mask Callback atkMode:
      | AM_MaskEnables = get_param(gcb, 'MaskEnables');
      | switch get_param(gcb, 'atkMode');
      |     case 'No attack'
      |         AM_MaskEnables{3} = 'off';
      |         AM_MaskEnables{4} = 'off';
      |     case 'Step attack'
      |         AM_MaskEnables{3} = 'on';
      |         AM_MaskEnables{4} = 'off';
      |     otherwise
      |         AM_MaskEnables{3} = 'on';
      |         AM_MaskEnables{4} = 'on';
      | end
      | set_param(gcb, 'MaskEnables', AM_MaskEnables);
      | 
      | clear AM_MaskEnables;
      mask Callback start:
      | SS_start = get_param(gcb, 'start');
      | if strcmp(SS_start, '') % empty
      |     set_param(gcb, 'start', '0');
      |     SS_start = 0;
      | end
      | SS_start = str2num(SS_start);
      | if isempty(SS_start)
      |     set_param(gcb, 'start', '0');
      |     SS_start = 0;
      |     warning('Parameter value must be a nimeric value.');
      | end
      | 
      | % set to the subsystem
      | set_param([gcb '/Attack Type Controller'], 'start', get_param(gcb, 'start'));
      | 
      | % get correct signal parameters
      | if strcmpi(get_param(gcb, 'switch_mode'),'custom attack')
      |     if ~exists_block([gcb '/SignalIn'])
      |         clear SS_start;
      |         return
      |     end
      |     % forward signal parameters if set
      |     SS_signal = get_param(gcb, 'signalin');
      |     if strcmp(SS_signal, '[]') || strcmp(SS_signal, '') % signal not set
      |         clear SS_signal;
      |         clear SS_start;
      |         return;
      |     else    % signal set
      |         SS_signal = evalin('base', SS_signal);
      |         SS_stime = str2num(get_param(gcb, 'stime'));
      |         if isempty(SS_stime) || SS_stime < -1 || (SS_stime < 0 && SS_stime > -1)
      |             clear SS_signal;
      |             clear SS_start;
      |             set_param(gcb, 'stime', '-1');
      |             SS_stime = -1;
      |             warning('Sample time must be a positve double or -1 for inherited value.')
      |         end
      | 
      |         if SS_stime == 0 || SS_stime == -1
      |             SS_stime = evalin('base', 'Ts_base');
      |         end
      | 
      | 
      |         signalstruct.time = SS_start:SS_stime:(SS_stime*(length(SS_signal) - 1) + SS_start);
      |         signalstruct.signals.values = SS_signal;
      | 
      | 		if strcmp(get_param(gcb, 'afterend'), 'Cyclic repetition')
      | 			SS_end = str2double(get_param(gcr, 'StopTime'));
      | 			while signalstruct.time(end) < SS_end
      | 				signalstruct.signals.values = [signalstruct.signals.values signalstruct.signals.values];
      | 				signalstruct.time = [signalstruct.time signalstruct.time+(signalstruct.time(end)-signalstruct.time(1))];
      | 			end
      | 		end
      | 
      | 		signalstruct.signals.values = signalstruct.signals.values(:);
      | 		signalstruct.time = signalstruct.time(:);
      |         %assignin('base', 'signalstruct', signalstruct)
      |         set_param([gcb '/SignalIn'], 'VariableName', 'signalstruct');
      | 		clear SS_signal;
      | 		clear SS_start;
      | 		clear SS_stime;
      | 		clear SS_end;
      |     end
      | 
      | end
      mask TypeOptions duration: Attack Type Controller/duration
      mask TypeOptions Value: Integrity attack value/Value
      mask Callback signalin:
      | if ~exists_block([gcb '/SignalIn'])
      |     return;
      | end
      | 
      | % forward signal parameters if set
      | SI_signal = get_param(gcb, 'signalin');
      | if strcmp(SI_signal, '[]') || strcmp(SI_signal, '') % signal not set
      |     set_param([gcb '/SignalIn'], 'VariableName', '[]');
      |     set_param(gcb, 'signalin', '[]');
      |     clear SI_signal;
      | else
      |     if ~exist(SI_signal)
      |         set_param(gcb, 'signalin', '[]');
      |         set_param([gcb '/SignalIn'], 'VariableName', '[]');
      |         warning('VAC:AttackController:Signal variable', ['Variable ' SI_signal ' not found.']);
      |         clear SI_signal;
      |         return;
      |     end
      | 
      |     SI_signal = evalin('base', SI_signal);
      |     if ~isvector(SI_signal)
      |         set_param(gcb, 'signalin', '[]');
      |         set_param([gcb '/SignalIn'], 'VariableName', '[]');
      |         warning('VAC:AttackController:Signal variable', ['Variable ' SI_signal ' must be a vector.']);
      |         clear SI_signal;
      |         return;
      |     end
      | 
      |     SI_stime = str2num(get_param(gcb, 'stime'));
      |     if isempty(SI_stime) || SI_stime < -1 || (SI_stime < 0 && SI_stime > -1)
      |         set_param(gcb, 'stime', '-1');
      |         SI_stime = -1;
      |         warning('VAC:AttackController:Signal variable', 'Sample time must be a positive double or -1 for inherited value.');
      |     end
      | 
      |     if SI_stime == 0 || SI_stime == -1
      |         SI_stime = evalin('base', 'Ts_base');
      |     end
      | 
      | 	SI_start = str2double(get_param(gcb, 'start'));
      | 	SI_start = SI_stime * ceil(SI_start/SI_stime);
      | 	signalstruct.time = SI_start:SI_stime:(SI_stime*(length(SI_signal) - 1) + SI_start);
      | 	signalstruct.signals.values = SI_signal;
      | 
      |     if strcmp(get_param(gcb, 'afterend'), 'Cyclic repetition')
      | 		SI_end = str2double(get_param(gcr, 'StopTime'));
      | 		while signalstruct.time(end) < SI_end
      | 			signalstruct.signals.values = [signalstruct.signals.values signalstruct.signals.values];
      | 			signalstruct.time = [signalstruct.time signalstruct.time+(signalstruct.time(end)-signalstruct.time(1))];
      | 		end
      | 	end
      | 
      | 	signalstruct.signals.values = signalstruct.signals.values(:);
      | 	signalstruct.time = signalstruct.time(:);
      |     %assignin('base', 'signalstruct', signalstruct)
      |     set_param([gcb '/SignalIn'], 'VariableName', 'signalstruct');
      | 	clear SI_stime;
      | 	clear SI_start;
      | 	clear SI_signal;
      | 	clear SI_end;
      | end
      mask Callback stime:
      | SQ_stime = get_param(gcb, 'stime');
      | if strcmp(SQ_stime, '') % empty
      |     set_param(gcb, 'stime', '-1');
      |     SQ_stime = -1;
      | end
      | SQ_stime = str2num(SQ_stime);
      | if isempty(SQ_stime)
      |     set_param(gcb, 'stime', '-1');
      |     SQ_stime = -1;
      |     warning('VAC:AttackController:Sample time','Sample time must be a positve double or -1 for inherited value.')
      | end
      | 
      | % get correct signal parameters
      | if strcmpi(get_param(gcb, 'switch_mode'),'custom attack')
      |     if ~exists_block([gcb '/SignalIn'])
      |         clear SS_start;
      |         return
      |     end
      |     % forward signal parameters if set
      |     SQ_signal = get_param(gcb, 'signalin');
      |     if strcmp(SQ_signal, '[]') || strcmp(SQ_signal, '') % signal not set
      |         clear SQ_signal;
      |         clear SQ_stime;
      |         return;
      |     else    % signal set
      |         SQ_signal = evalin('base', SQ_signal);
      |         if SQ_stime == 0 || SQ_stime == -1
      |             SQ_stime = evalin('base', 'Ts_base');
      |         end
      | 
      | 		SQ_start = str2double(get_param(gcb, 'start'));
      | 		SQ_start = SQ_stime * ceil(SQ_start/SQ_stime);
      | 		signalstruct.time = SQ_start:SQ_stime:(SQ_stime*(length(SQ_signal) - 1) + SQ_start);
      |         signalstruct.signals.values = SQ_signal;
      | 
      | 		if strcmp(get_param(gcb, 'afterend'), 'Cyclic repetition')
      | 			SQ_end = str2double(get_param(gcr, 'StopTime'));
      | 			while signalstruct.time(end) < SQ_end
      | 				signalstruct.signals.values = [signalstruct.signals.values signalstruct.signals.values];
      | 				signalstruct.time = [signalstruct.time signalstruct.time+(signalstruct.time(end)-signalstruct.time(1))];
      | 			end
      | 		end
      | 
      | 		signalstruct.signals.values = signalstruct.signals.values(:);
      | 		signalstruct.time = signalstruct.time(:);
      |         %assignin('base', 'signalstruct', signalstruct)
      |         set_param([gcb '/SignalIn'], 'VariableName', 'signalstruct');
      |     end
      | 	clear SQ_signal;
      | 	clear SQ_start;
      | 	clear SQ_stime;
      | 	clear SQ_end;
      | end
      mask TypeOptions afterend: Extrapolation | Setting to zero | Holding final value | Cyclic repetition
      mask Callback afterend:
      | if ~exists_block([gcb '/SignalIn'])
      |     return
      | end
      | 
      | % forward choosen value
      | if ~strcmp(get_param(gcb, 'afterend'), 'Cyclic repetition')
      | 	set_param([gcb '/SignalIn'], 'OutputAfterFinalValue', get_param(gcb, 'afterend'));
      | end
      | 
      | % forward signal parameters if set
      | SA_signal = get_param(gcb, 'signalin');
      | if strcmp(SA_signal, '[]') || strcmp(SA_signal, '') % signal not set
      |     set_param([gcb '/SignalIn'], 'VariableName', '[]');
      |     set_param(gcb, 'signalin', '[]');
      |     clear SA_signal;
      | else
      |     if ~exist(SA_signal)
      |         set_param(gcb, 'signalin', '[]');
      |         set_param([gcb '/SignalIn'], 'VariableName', '[]');
      |         warning('VAC:AttackController:After end', ['Variable ' SA_signal ' not found.']);
      |         clear SA_signal;
      |         return;
      |     end
      | 
      |     SA_signal = evalin('base', SA_signal);
      |     if ~isvector(SA_signal)
      |         set_param(gcb, 'signalin', '[]');
      |         set_param([gcb '/SignalIn'], 'VariableName', '[]');
      |         warning('VAC:AttackController:After end', ['Variable ' SA_signal ' must be a vector.']);
      |         clear SA_signal;
      |         return;
      |     end
      | 
      |     SA_stime = str2num(get_param(gcb, 'stime'));
      |     if isempty(SA_stime) || SA_stime < -1 || (SA_stime < 0 && SA_stime > -1)
      |         set_param(gcb, 'stime', '-1');
      |         SA_stime = -1;
      |         warning('VAC:AttackController:After end', 'Sample time must be a positive double or -1 for inherited value.');
      |     end
      | 
      |     if SA_stime == 0 || SA_stime == -1
      |         SA_stime = evalin('base', 'Ts_base');
      |     end
      | 
      | 	SA_start = str2double(get_param(gcb, 'start'));
      | 	SA_start = SA_stime * ceil(SA_start/SA_stime);
      | 	signalstruct.time = SA_start:SA_stime:(SA_stime*(length(SA_signal) - 1) + SA_start);
      | 	signalstruct.signals.values = SA_signal;
      | 
      | 	if strcmp(get_param(gcb, 'afterend'), 'Cyclic repetition')
      | 		SA_end = str2double(get_param(gcr, 'StopTime'));
      | 		while signalstruct.time(end) < SA_end
      | 			signalstruct.signals.values = [signalstruct.signals.values signalstruct.signals.values];
      | 			signalstruct.time = [signalstruct.time signalstruct.time+(signalstruct.time(end)-signalstruct.time(1))];
      | 		end
      |     end
      | 
      |     signalstruct.time = signalstruct.time(:);
      | 	signalstruct.signals.values = signalstruct.signals.values(:);
      |     %assignin('base', 'signalstruct', signalstruct)
      |     set_param([gcb '/SignalIn'], 'VariableName', 'signalstruct');
      | 
      | 	clear SA_stime;
      | 	clear SA_start;
      | 	clear SA_signal;
      | 	clear SA_end;
      | end
      mask Display:
      | disp([get_param(gcb, 'switch_mode') '\n' get_param(gcb, 'atkMode')])
      | port_label('input', 1, 'signal in')
      | port_label('output', 1, 'signal out')
  xmeas42 attack controller : Subsystem  AncestorBlock=VAlib/Attack Controller  mask(Attack controller){switch_mode=Integrity attack, atkMode=No attack, start=1, duration=1, Value=0, signalin=[], stime=-1, afterend=Holding final value}
      mask prompts: switch_mode "Attack Type:"; atkMode "Attack Mode:"; Value "Integrity Attack Value:"; signalin "Signal variable:"; stime "Sample time:"; afterend "Output after final:"
      mask help:
      | Attack controller block controls an attack on choosen variable on the specified time.
      | Attack types: DoS, Integrity and custom signal attack.
      | Modes: Step attack on specified time, Interval to specified time, Periodic and no attack.
      mask TypeOptions switch_mode: Integrity attack | DOS attack | Custom attack
      mask Callback switch_mode:
      | SM_MaskEnables = get_param(gcb, 'MaskEnables');
      | switch get_param(gcb, 'switch_mode')
      |     case 'Integrity attack'
      |         set_param([gcb,'/Switch value'], 'Value', '1');
      |         SM_MaskEnables{5} = 'on';
      |         SM_MaskEnables{6} = 'off';
      |         SM_MaskEnables{7} = 'off';
      |         SM_MaskEnables{8} = 'off';
      |     case 'DOS attack'
      |         set_param([gcb,'/Switch value'], 'Value', '3');
      |         SM_MaskEnables{5} = 'off';
      |         SM_MaskEnables{6} = 'off';
      |         SM_MaskEnables{7} = 'off';
      |         SM_MaskEnables{8} = 'off';
      |     case 'Custom attack'
      |         set_param([gcb,'/Switch value'], 'Value', '2');
      |         SM_MaskEnables{5} = 'off';
      |         SM_MaskEnables{6} = 'on';
      |         SM_MaskEnables{7} = 'on';
      |         SM_MaskEnables{8} = 'on';
      | end
      | set_param(gcb,'MaskEnables',SM_MaskEnables);
      | clear SM_MaskEnables;
      | 
      | % creat or remove block for custom attack
      | if strcmpi(get_param(gcb, 'switch_mode'), 'Custom attack') && ~exists_block([gcb '/SignalIn']) % creat block
      |     if exists_block([gcb, '/ReplaceBlock']);
      |         delete_line(gcb, 'ReplaceBlock/1', 'Multiport Switch/3');
      |         delete_block([gcb '/ReplaceBlock']);
      |     end
      | 
      |     add_block('built-in/FromWorkspace', [gcb '/SignalIn'], 'Position', [50 400 120 430]);
      |     add_line(gcb, 'SignalIn/1', 'Multiport Switch/3', 'autorouting', 'on');
      |     %set params
      |     set_param([gcb '/SignalIn'], 'SampleTime', '0');
      |     %set_param([gcb '/SignalIn'], 'VariableName', '[]');
      |     set_param([gcb '/SignalIn'], 'Interpolate', 'on');
      |     set_param([gcb '/SignalIn'], 'ZeroCross', 'off');
      |     %set_param([gcb '/' name], 'OutputAfterFinalValue', 'Setting to zero');
      |     %set_param([gcb '/' name], 'OutputAfterFinalValue', 'Cyclic repetition');
      |     %set_param([gcb '/' name], 'OutputAfterFinalValue', 'Extrapolation');
      |     %set_param([gcb '/' name], 'OutputAfterFinalValue', 'Holding final value');
      | 
      |     % forward signal parameters if set
      |     SW_signal = get_param(gcb, 'signalin');
      |     if strcmp(SW_signal, '[]') || strcmp(SW_signal, '') % signal not set
      |         set_param(gcb, 'signalin', '[]');
      |         set_param([gcb '/SignalIn'], 'VariableName', '[]');
      |         clear SW_signal;
      |         return;
      |     else    % signal set
      |         % check signal
      |         if ~exist(SW_signal)
      |             set_param(gcb, 'signalin', '[]');
      |             set_param([gcb '/SignalIn'], 'VariableName', '[]');
      |             warning(['Variable ' SW_signal ' not found.']);
      |             clear SW_signal;
      |             return;
      |         end
      |         SW_signal = evalin('base', SW_signal);
      |         if ~isvector(SW_signal)
      |             set_param(gcb, 'signalin', '');
      |             set_param([gcb '/SignalIn'], 'VariableName', '[]');
      |             warning(['Variable ' SW_signal ' must be a vector.']);
      |             clear SW_signal;
      |             return;
      |         end
      |         SW_stime = str2num(get_param(gcb, 'stime'));
      |         if isempty(SW_stime) || SW_stime < -1 || (SW_stime < 0 && SW_stime > -1)
      |             set_param(gcb, 'stime', '-1');
      |             SW_stime = -1;
      |             warning('Sample time must be a positive double or -1 for inherited value.');
      |         end
      | 
      |         if SW_stime == 0 || SW_stime == -1
      |             SW_stime = evalin('base', 'Ts_base');
      |         end
      | 
      |         SW_start = str2num(get_param(gcb, 'start'));
      |         SW_start = SW_stime * ceil(SW_start/SW_stime);
      |         signalstruct.time = SW_start:SW_stime:(SW_stime*(length(SW_signal) - 1) + SW_start);
      |         signalstruct.signals.values = SW_signal;
      | 
      | 		if strcmp(get_param(gcb, 'afterend'), 'Cyclic repetition')
      | 			SW_end = str2double(get_param(gcr, 'StopTime'));
      | 			while signalstruct.time(end) < SW_end
      | 				signalstruct.signals.values = [signalstruct.signals.values signalstruct.signals.values];
      | 				signalstruct.time = [signalstruct.time signalstruct.time+(signalstruct.time(end)-signalstruct.time(1))];
      | 			end
      | 		end
      | 
      | 		signalstruct.signals.values = signalstruct.signals.values(:);
      | 		signalstruct.time = signalstruct.time(:);
      |         %assignin('base', 'signalstruct', signalstruct)
      |         set_param([gcb '/SignalIn'], 'VariableName', 'signalstruct');
      |     end
      | 
      |     clear SW_signal;
      | 	clear SW_start;
      |     clear SW_stime;
      | 	clear SW_end;
      | elseif ~strcmpi(get_param(gcb, 'switch_mode'), 'Custom attack') && exists_block([gcb '/SignalIn']) % delete block
      |     delete_line(gcb, 'SignalIn/1', 'Multiport Switch/3');
      |     delete_block([gcb '/SignalIn']);
      |     % replace with constant value
      |     add_block(['built-in/Constant'], [gcb '/ReplaceBlock'], 'Position', [50 400 120 430]);
      |     add_line(gcb, ['ReplaceBlock/1'], 'Multiport Switch/3', 'autorouting', 'on');
      | end
      mask TypeOptions atkMode: Attack Type Controller/atkMode
      mask Callback atkMode:
      | AM_MaskEnables = get_param(gcb, 'MaskEnables');
      | switch get_param(gcb, 'atkMode');
      |     case 'No attack'
      |         AM_MaskEnables{3} = 'off';
      |         AM_MaskEnables{4} = 'off';
      |     case 'Step attack'
      |         AM_MaskEnables{3} = 'on';
      |         AM_MaskEnables{4} = 'off';
      |     otherwise
      |         AM_MaskEnables{3} = 'on';
      |         AM_MaskEnables{4} = 'on';
      | end
      | set_param(gcb, 'MaskEnables', AM_MaskEnables);
      | 
      | clear AM_MaskEnables;
      mask Callback start:
      | SS_start = get_param(gcb, 'start');
      | if strcmp(SS_start, '') % empty
      |     set_param(gcb, 'start', '0');
      |     SS_start = 0;
      | end
      | SS_start = str2num(SS_start);
      | if isempty(SS_start)
      |     set_param(gcb, 'start', '0');
      |     SS_start = 0;
      |     warning('Parameter value must be a nimeric value.');
      | end
      | 
      | % set to the subsystem
      | set_param([gcb '/Attack Type Controller'], 'start', get_param(gcb, 'start'));
      | 
      | % get correct signal parameters
      | if strcmpi(get_param(gcb, 'switch_mode'),'custom attack')
      |     if ~exists_block([gcb '/SignalIn'])
      |         clear SS_start;
      |         return
      |     end
      |     % forward signal parameters if set
      |     SS_signal = get_param(gcb, 'signalin');
      |     if strcmp(SS_signal, '[]') || strcmp(SS_signal, '') % signal not set
      |         clear SS_signal;
      |         clear SS_start;
      |         return;
      |     else    % signal set
      |         SS_signal = evalin('base', SS_signal);
      |         SS_stime = str2num(get_param(gcb, 'stime'));
      |         if isempty(SS_stime) || SS_stime < -1 || (SS_stime < 0 && SS_stime > -1)
      |             clear SS_signal;
      |             clear SS_start;
      |             set_param(gcb, 'stime', '-1');
      |             SS_stime = -1;
      |             warning('Sample time must be a positve double or -1 for inherited value.')
      |         end
      | 
      |         if SS_stime == 0 || SS_stime == -1
      |             SS_stime = evalin('base', 'Ts_base');
      |         end
      | 
      | 
      |         signalstruct.time = SS_start:SS_stime:(SS_stime*(length(SS_signal) - 1) + SS_start);
      |         signalstruct.signals.values = SS_signal;
      | 
      | 		if strcmp(get_param(gcb, 'afterend'), 'Cyclic repetition')
      | 			SS_end = str2double(get_param(gcr, 'StopTime'));
      | 			while signalstruct.time(end) < SS_end
      | 				signalstruct.signals.values = [signalstruct.signals.values signalstruct.signals.values];
      | 				signalstruct.time = [signalstruct.time signalstruct.time+(signalstruct.time(end)-signalstruct.time(1))];
      | 			end
      | 		end
      | 
      | 		signalstruct.signals.values = signalstruct.signals.values(:);
      | 		signalstruct.time = signalstruct.time(:);
      |         %assignin('base', 'signalstruct', signalstruct)
      |         set_param([gcb '/SignalIn'], 'VariableName', 'signalstruct');
      | 		clear SS_signal;
      | 		clear SS_start;
      | 		clear SS_stime;
      | 		clear SS_end;
      |     end
      | 
      | end
      mask TypeOptions duration: Attack Type Controller/duration
      mask TypeOptions Value: Integrity attack value/Value
      mask Callback signalin:
      | if ~exists_block([gcb '/SignalIn'])
      |     return;
      | end
      | 
      | % forward signal parameters if set
      | SI_signal = get_param(gcb, 'signalin');
      | if strcmp(SI_signal, '[]') || strcmp(SI_signal, '') % signal not set
      |     set_param([gcb '/SignalIn'], 'VariableName', '[]');
      |     set_param(gcb, 'signalin', '[]');
      |     clear SI_signal;
      | else
      |     if ~exist(SI_signal)
      |         set_param(gcb, 'signalin', '[]');
      |         set_param([gcb '/SignalIn'], 'VariableName', '[]');
      |         warning('VAC:AttackController:Signal variable', ['Variable ' SI_signal ' not found.']);
      |         clear SI_signal;
      |         return;
      |     end
      | 
      |     SI_signal = evalin('base', SI_signal);
      |     if ~isvector(SI_signal)
      |         set_param(gcb, 'signalin', '[]');
      |         set_param([gcb '/SignalIn'], 'VariableName', '[]');
      |         warning('VAC:AttackController:Signal variable', ['Variable ' SI_signal ' must be a vector.']);
      |         clear SI_signal;
      |         return;
      |     end
      | 
      |     SI_stime = str2num(get_param(gcb, 'stime'));
      |     if isempty(SI_stime) || SI_stime < -1 || (SI_stime < 0 && SI_stime > -1)
      |         set_param(gcb, 'stime', '-1');
      |         SI_stime = -1;
      |         warning('VAC:AttackController:Signal variable', 'Sample time must be a positive double or -1 for inherited value.');
      |     end
      | 
      |     if SI_stime == 0 || SI_stime == -1
      |         SI_stime = evalin('base', 'Ts_base');
      |     end
      | 
      | 	SI_start = str2double(get_param(gcb, 'start'));
      | 	SI_start = SI_stime * ceil(SI_start/SI_stime);
      | 	signalstruct.time = SI_start:SI_stime:(SI_stime*(length(SI_signal) - 1) + SI_start);
      | 	signalstruct.signals.values = SI_signal;
      | 
      |     if strcmp(get_param(gcb, 'afterend'), 'Cyclic repetition')
      | 		SI_end = str2double(get_param(gcr, 'StopTime'));
      | 		while signalstruct.time(end) < SI_end
      | 			signalstruct.signals.values = [signalstruct.signals.values signalstruct.signals.values];
      | 			signalstruct.time = [signalstruct.time signalstruct.time+(signalstruct.time(end)-signalstruct.time(1))];
      | 		end
      | 	end
      | 
      | 	signalstruct.signals.values = signalstruct.signals.values(:);
      | 	signalstruct.time = signalstruct.time(:);
      |     %assignin('base', 'signalstruct', signalstruct)
      |     set_param([gcb '/SignalIn'], 'VariableName', 'signalstruct');
      | 	clear SI_stime;
      | 	clear SI_start;
      | 	clear SI_signal;
      | 	clear SI_end;
      | end
      mask Callback stime:
      | SQ_stime = get_param(gcb, 'stime');
      | if strcmp(SQ_stime, '') % empty
      |     set_param(gcb, 'stime', '-1');
      |     SQ_stime = -1;
      | end
      | SQ_stime = str2num(SQ_stime);
      | if isempty(SQ_stime)
      |     set_param(gcb, 'stime', '-1');
      |     SQ_stime = -1;
      |     warning('VAC:AttackController:Sample time','Sample time must be a positve double or -1 for inherited value.')
      | end
      | 
      | % get correct signal parameters
      | if strcmpi(get_param(gcb, 'switch_mode'),'custom attack')
      |     if ~exists_block([gcb '/SignalIn'])
      |         clear SS_start;
      |         return
      |     end
      |     % forward signal parameters if set
      |     SQ_signal = get_param(gcb, 'signalin');
      |     if strcmp(SQ_signal, '[]') || strcmp(SQ_signal, '') % signal not set
      |         clear SQ_signal;
      |         clear SQ_stime;
      |         return;
      |     else    % signal set
      |         SQ_signal = evalin('base', SQ_signal);
      |         if SQ_stime == 0 || SQ_stime == -1
      |             SQ_stime = evalin('base', 'Ts_base');
      |         end
      | 
      | 		SQ_start = str2double(get_param(gcb, 'start'));
      | 		SQ_start = SQ_stime * ceil(SQ_start/SQ_stime);
      | 		signalstruct.time = SQ_start:SQ_stime:(SQ_stime*(length(SQ_signal) - 1) + SQ_start);
      |         signalstruct.signals.values = SQ_signal;
      | 
      | 		if strcmp(get_param(gcb, 'afterend'), 'Cyclic repetition')
      | 			SQ_end = str2double(get_param(gcr, 'StopTime'));
      | 			while signalstruct.time(end) < SQ_end
      | 				signalstruct.signals.values = [signalstruct.signals.values signalstruct.signals.values];
      | 				signalstruct.time = [signalstruct.time signalstruct.time+(signalstruct.time(end)-signalstruct.time(1))];
      | 			end
      | 		end
      | 
      | 		signalstruct.signals.values = signalstruct.signals.values(:);
      | 		signalstruct.time = signalstruct.time(:);
      |         %assignin('base', 'signalstruct', signalstruct)
      |         set_param([gcb '/SignalIn'], 'VariableName', 'signalstruct');
      |     end
      | 	clear SQ_signal;
      | 	clear SQ_start;
      | 	clear SQ_stime;
      | 	clear SQ_end;
      | end
      mask TypeOptions afterend: Extrapolation | Setting to zero | Holding final value | Cyclic repetition
      mask Callback afterend:
      | if ~exists_block([gcb '/SignalIn'])
      |     return
      | end
      | 
      | % forward choosen value
      | if ~strcmp(get_param(gcb, 'afterend'), 'Cyclic repetition')
      | 	set_param([gcb '/SignalIn'], 'OutputAfterFinalValue', get_param(gcb, 'afterend'));
      | end
      | 
      | % forward signal parameters if set
      | SA_signal = get_param(gcb, 'signalin');
      | if strcmp(SA_signal, '[]') || strcmp(SA_signal, '') % signal not set
      |     set_param([gcb '/SignalIn'], 'VariableName', '[]');
      |     set_param(gcb, 'signalin', '[]');
      |     clear SA_signal;
      | else
      |     if ~exist(SA_signal)
      |         set_param(gcb, 'signalin', '[]');
      |         set_param([gcb '/SignalIn'], 'VariableName', '[]');
      |         warning('VAC:AttackController:After end', ['Variable ' SA_signal ' not found.']);
      |         clear SA_signal;
      |         return;
      |     end
      | 
      |     SA_signal = evalin('base', SA_signal);
      |     if ~isvector(SA_signal)
      |         set_param(gcb, 'signalin', '[]');
      |         set_param([gcb '/SignalIn'], 'VariableName', '[]');
      |         warning('VAC:AttackController:After end', ['Variable ' SA_signal ' must be a vector.']);
      |         clear SA_signal;
      |         return;
      |     end
      | 
      |     SA_stime = str2num(get_param(gcb, 'stime'));
      |     if isempty(SA_stime) || SA_stime < -1 || (SA_stime < 0 && SA_stime > -1)
      |         set_param(gcb, 'stime', '-1');
      |         SA_stime = -1;
      |         warning('VAC:AttackController:After end', 'Sample time must be a positive double or -1 for inherited value.');
      |     end
      | 
      |     if SA_stime == 0 || SA_stime == -1
      |         SA_stime = evalin('base', 'Ts_base');
      |     end
      | 
      | 	SA_start = str2double(get_param(gcb, 'start'));
      | 	SA_start = SA_stime * ceil(SA_start/SA_stime);
      | 	signalstruct.time = SA_start:SA_stime:(SA_stime*(length(SA_signal) - 1) + SA_start);
      | 	signalstruct.signals.values = SA_signal;
      | 
      | 	if strcmp(get_param(gcb, 'afterend'), 'Cyclic repetition')
      | 		SA_end = str2double(get_param(gcr, 'StopTime'));
      | 		while signalstruct.time(end) < SA_end
      | 			signalstruct.signals.values = [signalstruct.signals.values signalstruct.signals.values];
      | 			signalstruct.time = [signalstruct.time signalstruct.time+(signalstruct.time(end)-signalstruct.time(1))];
      | 		end
      |     end
      | 
      |     signalstruct.time = signalstruct.time(:);
      | 	signalstruct.signals.values = signalstruct.signals.values(:);
      |     %assignin('base', 'signalstruct', signalstruct)
      |     set_param([gcb '/SignalIn'], 'VariableName', 'signalstruct');
      | 
      | 	clear SA_stime;
      | 	clear SA_start;
      | 	clear SA_signal;
      | 	clear SA_end;
      | end
      mask Display:
      | disp([get_param(gcb, 'switch_mode') '\n' get_param(gcb, 'atkMode')])
      | port_label('input', 1, 'signal in')
      | port_label('output', 1, 'signal out')
  xmeas43 attack controller : Subsystem  AncestorBlock=VAlib/Attack Controller  mask(Attack controller){switch_mode=Integrity attack, atkMode=No attack, start=1, duration=1, Value=0, signalin=[], stime=-1, afterend=Holding final value}
      mask prompts: switch_mode "Attack Type:"; atkMode "Attack Mode:"; Value "Integrity Attack Value:"; signalin "Signal variable:"; stime "Sample time:"; afterend "Output after final:"
      mask help:
      | Attack controller block controls an attack on choosen variable on the specified time.
      | Attack types: DoS, Integrity and custom signal attack.
      | Modes: Step attack on specified time, Interval to specified time, Periodic and no attack.
      mask TypeOptions switch_mode: Integrity attack | DOS attack | Custom attack
      mask Callback switch_mode:
      | SM_MaskEnables = get_param(gcb, 'MaskEnables');
      | switch get_param(gcb, 'switch_mode')
      |     case 'Integrity attack'
      |         set_param([gcb,'/Switch value'], 'Value', '1');
      |         SM_MaskEnables{5} = 'on';
      |         SM_MaskEnables{6} = 'off';
      |         SM_MaskEnables{7} = 'off';
      |         SM_MaskEnables{8} = 'off';
      |     case 'DOS attack'
      |         set_param([gcb,'/Switch value'], 'Value', '3');
      |         SM_MaskEnables{5} = 'off';
      |         SM_MaskEnables{6} = 'off';
      |         SM_MaskEnables{7} = 'off';
      |         SM_MaskEnables{8} = 'off';
      |     case 'Custom attack'
      |         set_param([gcb,'/Switch value'], 'Value', '2');
      |         SM_MaskEnables{5} = 'off';
      |         SM_MaskEnables{6} = 'on';
      |         SM_MaskEnables{7} = 'on';
      |         SM_MaskEnables{8} = 'on';
      | end
      | set_param(gcb,'MaskEnables',SM_MaskEnables);
      | clear SM_MaskEnables;
      | 
      | % creat or remove block for custom attack
      | if strcmpi(get_param(gcb, 'switch_mode'), 'Custom attack') && ~exists_block([gcb '/SignalIn']) % creat block
      |     if exists_block([gcb, '/ReplaceBlock']);
      |         delete_line(gcb, 'ReplaceBlock/1', 'Multiport Switch/3');
      |         delete_block([gcb '/ReplaceBlock']);
      |     end
      | 
      |     add_block('built-in/FromWorkspace', [gcb '/SignalIn'], 'Position', [50 400 120 430]);
      |     add_line(gcb, 'SignalIn/1', 'Multiport Switch/3', 'autorouting', 'on');
      |     %set params
      |     set_param([gcb '/SignalIn'], 'SampleTime', '0');
      |     %set_param([gcb '/SignalIn'], 'VariableName', '[]');
      |     set_param([gcb '/SignalIn'], 'Interpolate', 'on');
      |     set_param([gcb '/SignalIn'], 'ZeroCross', 'off');
      |     %set_param([gcb '/' name], 'OutputAfterFinalValue', 'Setting to zero');
      |     %set_param([gcb '/' name], 'OutputAfterFinalValue', 'Cyclic repetition');
      |     %set_param([gcb '/' name], 'OutputAfterFinalValue', 'Extrapolation');
      |     %set_param([gcb '/' name], 'OutputAfterFinalValue', 'Holding final value');
      | 
      |     % forward signal parameters if set
      |     SW_signal = get_param(gcb, 'signalin');
      |     if strcmp(SW_signal, '[]') || strcmp(SW_signal, '') % signal not set
      |         set_param(gcb, 'signalin', '[]');
      |         set_param([gcb '/SignalIn'], 'VariableName', '[]');
      |         clear SW_signal;
      |         return;
      |     else    % signal set
      |         % check signal
      |         if ~exist(SW_signal)
      |             set_param(gcb, 'signalin', '[]');
      |             set_param([gcb '/SignalIn'], 'VariableName', '[]');
      |             warning(['Variable ' SW_signal ' not found.']);
      |             clear SW_signal;
      |             return;
      |         end
      |         SW_signal = evalin('base', SW_signal);
      |         if ~isvector(SW_signal)
      |             set_param(gcb, 'signalin', '');
      |             set_param([gcb '/SignalIn'], 'VariableName', '[]');
      |             warning(['Variable ' SW_signal ' must be a vector.']);
      |             clear SW_signal;
      |             return;
      |         end
      |         SW_stime = str2num(get_param(gcb, 'stime'));
      |         if isempty(SW_stime) || SW_stime < -1 || (SW_stime < 0 && SW_stime > -1)
      |             set_param(gcb, 'stime', '-1');
      |             SW_stime = -1;
      |             warning('Sample time must be a positive double or -1 for inherited value.');
      |         end
      | 
      |         if SW_stime == 0 || SW_stime == -1
      |             SW_stime = evalin('base', 'Ts_base');
      |         end
      | 
      |         SW_start = str2num(get_param(gcb, 'start'));
      |         SW_start = SW_stime * ceil(SW_start/SW_stime);
      |         signalstruct.time = SW_start:SW_stime:(SW_stime*(length(SW_signal) - 1) + SW_start);
      |         signalstruct.signals.values = SW_signal;
      | 
      | 		if strcmp(get_param(gcb, 'afterend'), 'Cyclic repetition')
      | 			SW_end = str2double(get_param(gcr, 'StopTime'));
      | 			while signalstruct.time(end) < SW_end
      | 				signalstruct.signals.values = [signalstruct.signals.values signalstruct.signals.values];
      | 				signalstruct.time = [signalstruct.time signalstruct.time+(signalstruct.time(end)-signalstruct.time(1))];
      | 			end
      | 		end
      | 
      | 		signalstruct.signals.values = signalstruct.signals.values(:);
      | 		signalstruct.time = signalstruct.time(:);
      |         %assignin('base', 'signalstruct', signalstruct)
      |         set_param([gcb '/SignalIn'], 'VariableName', 'signalstruct');
      |     end
      | 
      |     clear SW_signal;
      | 	clear SW_start;
      |     clear SW_stime;
      | 	clear SW_end;
      | elseif ~strcmpi(get_param(gcb, 'switch_mode'), 'Custom attack') && exists_block([gcb '/SignalIn']) % delete block
      |     delete_line(gcb, 'SignalIn/1', 'Multiport Switch/3');
      |     delete_block([gcb '/SignalIn']);
      |     % replace with constant value
      |     add_block(['built-in/Constant'], [gcb '/ReplaceBlock'], 'Position', [50 400 120 430]);
      |     add_line(gcb, ['ReplaceBlock/1'], 'Multiport Switch/3', 'autorouting', 'on');
      | end
      mask TypeOptions atkMode: Attack Type Controller/atkMode
      mask Callback atkMode:
      | AM_MaskEnables = get_param(gcb, 'MaskEnables');
      | switch get_param(gcb, 'atkMode');
      |     case 'No attack'
      |         AM_MaskEnables{3} = 'off';
      |         AM_MaskEnables{4} = 'off';
      |     case 'Step attack'
      |         AM_MaskEnables{3} = 'on';
      |         AM_MaskEnables{4} = 'off';
      |     otherwise
      |         AM_MaskEnables{3} = 'on';
      |         AM_MaskEnables{4} = 'on';
      | end
      | set_param(gcb, 'MaskEnables', AM_MaskEnables);
      | 
      | clear AM_MaskEnables;
      mask Callback start:
      | SS_start = get_param(gcb, 'start');
      | if strcmp(SS_start, '') % empty
      |     set_param(gcb, 'start', '0');
      |     SS_start = 0;
      | end
      | SS_start = str2num(SS_start);
      | if isempty(SS_start)
      |     set_param(gcb, 'start', '0');
      |     SS_start = 0;
      |     warning('Parameter value must be a nimeric value.');
      | end
      | 
      | % set to the subsystem
      | set_param([gcb '/Attack Type Controller'], 'start', get_param(gcb, 'start'));
      | 
      | % get correct signal parameters
      | if strcmpi(get_param(gcb, 'switch_mode'),'custom attack')
      |     if ~exists_block([gcb '/SignalIn'])
      |         clear SS_start;
      |         return
      |     end
      |     % forward signal parameters if set
      |     SS_signal = get_param(gcb, 'signalin');
      |     if strcmp(SS_signal, '[]') || strcmp(SS_signal, '') % signal not set
      |         clear SS_signal;
      |         clear SS_start;
      |         return;
      |     else    % signal set
      |         SS_signal = evalin('base', SS_signal);
      |         SS_stime = str2num(get_param(gcb, 'stime'));
      |         if isempty(SS_stime) || SS_stime < -1 || (SS_stime < 0 && SS_stime > -1)
      |             clear SS_signal;
      |             clear SS_start;
      |             set_param(gcb, 'stime', '-1');
      |             SS_stime = -1;
      |             warning('Sample time must be a positve double or -1 for inherited value.')
      |         end
      | 
      |         if SS_stime == 0 || SS_stime == -1
      |             SS_stime = evalin('base', 'Ts_base');
      |         end
      | 
      | 
      |         signalstruct.time = SS_start:SS_stime:(SS_stime*(length(SS_signal) - 1) + SS_start);
      |         signalstruct.signals.values = SS_signal;
      | 
      | 		if strcmp(get_param(gcb, 'afterend'), 'Cyclic repetition')
      | 			SS_end = str2double(get_param(gcr, 'StopTime'));
      | 			while signalstruct.time(end) < SS_end
      | 				signalstruct.signals.values = [signalstruct.signals.values signalstruct.signals.values];
      | 				signalstruct.time = [signalstruct.time signalstruct.time+(signalstruct.time(end)-signalstruct.time(1))];
      | 			end
      | 		end
      | 
      | 		signalstruct.signals.values = signalstruct.signals.values(:);
      | 		signalstruct.time = signalstruct.time(:);
      |         %assignin('base', 'signalstruct', signalstruct)
      |         set_param([gcb '/SignalIn'], 'VariableName', 'signalstruct');
      | 		clear SS_signal;
      | 		clear SS_start;
      | 		clear SS_stime;
      | 		clear SS_end;
      |     end
      | 
      | end
      mask TypeOptions duration: Attack Type Controller/duration
      mask TypeOptions Value: Integrity attack value/Value
      mask Callback signalin:
      | if ~exists_block([gcb '/SignalIn'])
      |     return;
      | end
      | 
      | % forward signal parameters if set
      | SI_signal = get_param(gcb, 'signalin');
      | if strcmp(SI_signal, '[]') || strcmp(SI_signal, '') % signal not set
      |     set_param([gcb '/SignalIn'], 'VariableName', '[]');
      |     set_param(gcb, 'signalin', '[]');
      |     clear SI_signal;
      | else
      |     if ~exist(SI_signal)
      |         set_param(gcb, 'signalin', '[]');
      |         set_param([gcb '/SignalIn'], 'VariableName', '[]');
      |         warning('VAC:AttackController:Signal variable', ['Variable ' SI_signal ' not found.']);
      |         clear SI_signal;
      |         return;
      |     end
      | 
      |     SI_signal = evalin('base', SI_signal);
      |     if ~isvector(SI_signal)
      |         set_param(gcb, 'signalin', '[]');
      |         set_param([gcb '/SignalIn'], 'VariableName', '[]');
      |         warning('VAC:AttackController:Signal variable', ['Variable ' SI_signal ' must be a vector.']);
      |         clear SI_signal;
      |         return;
      |     end
      | 
      |     SI_stime = str2num(get_param(gcb, 'stime'));
      |     if isempty(SI_stime) || SI_stime < -1 || (SI_stime < 0 && SI_stime > -1)
      |         set_param(gcb, 'stime', '-1');
      |         SI_stime = -1;
      |         warning('VAC:AttackController:Signal variable', 'Sample time must be a positive double or -1 for inherited value.');
      |     end
      | 
      |     if SI_stime == 0 || SI_stime == -1
      |         SI_stime = evalin('base', 'Ts_base');
      |     end
      | 
      | 	SI_start = str2double(get_param(gcb, 'start'));
      | 	SI_start = SI_stime * ceil(SI_start/SI_stime);
      | 	signalstruct.time = SI_start:SI_stime:(SI_stime*(length(SI_signal) - 1) + SI_start);
      | 	signalstruct.signals.values = SI_signal;
      | 
      |     if strcmp(get_param(gcb, 'afterend'), 'Cyclic repetition')
      | 		SI_end = str2double(get_param(gcr, 'StopTime'));
      | 		while signalstruct.time(end) < SI_end
      | 			signalstruct.signals.values = [signalstruct.signals.values signalstruct.signals.values];
      | 			signalstruct.time = [signalstruct.time signalstruct.time+(signalstruct.time(end)-signalstruct.time(1))];
      | 		end
      | 	end
      | 
      | 	signalstruct.signals.values = signalstruct.signals.values(:);
      | 	signalstruct.time = signalstruct.time(:);
      |     %assignin('base', 'signalstruct', signalstruct)
      |     set_param([gcb '/SignalIn'], 'VariableName', 'signalstruct');
      | 	clear SI_stime;
      | 	clear SI_start;
      | 	clear SI_signal;
      | 	clear SI_end;
      | end
      mask Callback stime:
      | SQ_stime = get_param(gcb, 'stime');
      | if strcmp(SQ_stime, '') % empty
      |     set_param(gcb, 'stime', '-1');
      |     SQ_stime = -1;
      | end
      | SQ_stime = str2num(SQ_stime);
      | if isempty(SQ_stime)
      |     set_param(gcb, 'stime', '-1');
      |     SQ_stime = -1;
      |     warning('VAC:AttackController:Sample time','Sample time must be a positve double or -1 for inherited value.')
      | end
      | 
      | % get correct signal parameters
      | if strcmpi(get_param(gcb, 'switch_mode'),'custom attack')
      |     if ~exists_block([gcb '/SignalIn'])
      |         clear SS_start;
      |         return
      |     end
      |     % forward signal parameters if set
      |     SQ_signal = get_param(gcb, 'signalin');
      |     if strcmp(SQ_signal, '[]') || strcmp(SQ_signal, '') % signal not set
      |         clear SQ_signal;
      |         clear SQ_stime;
      |         return;
      |     else    % signal set
      |         SQ_signal = evalin('base', SQ_signal);
      |         if SQ_stime == 0 || SQ_stime == -1
      |             SQ_stime = evalin('base', 'Ts_base');
      |         end
      | 
      | 		SQ_start = str2double(get_param(gcb, 'start'));
      | 		SQ_start = SQ_stime * ceil(SQ_start/SQ_stime);
      | 		signalstruct.time = SQ_start:SQ_stime:(SQ_stime*(length(SQ_signal) - 1) + SQ_start);
      |         signalstruct.signals.values = SQ_signal;
      | 
      | 		if strcmp(get_param(gcb, 'afterend'), 'Cyclic repetition')
      | 			SQ_end = str2double(get_param(gcr, 'StopTime'));
      | 			while signalstruct.time(end) < SQ_end
      | 				signalstruct.signals.values = [signalstruct.signals.values signalstruct.signals.values];
      | 				signalstruct.time = [signalstruct.time signalstruct.time+(signalstruct.time(end)-signalstruct.time(1))];
      | 			end
      | 		end
      | 
      | 		signalstruct.signals.values = signalstruct.signals.values(:);
      | 		signalstruct.time = signalstruct.time(:);
      |         %assignin('base', 'signalstruct', signalstruct)
      |         set_param([gcb '/SignalIn'], 'VariableName', 'signalstruct');
      |     end
      | 	clear SQ_signal;
      | 	clear SQ_start;
      | 	clear SQ_stime;
      | 	clear SQ_end;
      | end
      mask TypeOptions afterend: Extrapolation | Setting to zero | Holding final value | Cyclic repetition
      mask Callback afterend:
      | if ~exists_block([gcb '/SignalIn'])
      |     return
      | end
      | 
      | % forward choosen value
      | if ~strcmp(get_param(gcb, 'afterend'), 'Cyclic repetition')
      | 	set_param([gcb '/SignalIn'], 'OutputAfterFinalValue', get_param(gcb, 'afterend'));
      | end
      | 
      | % forward signal parameters if set
      | SA_signal = get_param(gcb, 'signalin');
      | if strcmp(SA_signal, '[]') || strcmp(SA_signal, '') % signal not set
      |     set_param([gcb '/SignalIn'], 'VariableName', '[]');
      |     set_param(gcb, 'signalin', '[]');
      |     clear SA_signal;
      | else
      |     if ~exist(SA_signal)
      |         set_param(gcb, 'signalin', '[]');
      |         set_param([gcb '/SignalIn'], 'VariableName', '[]');
      |         warning('VAC:AttackController:After end', ['Variable ' SA_signal ' not found.']);
      |         clear SA_signal;
      |         return;
      |     end
      | 
      |     SA_signal = evalin('base', SA_signal);
      |     if ~isvector(SA_signal)
      |         set_param(gcb, 'signalin', '[]');
      |         set_param([gcb '/SignalIn'], 'VariableName', '[]');
      |         warning('VAC:AttackController:After end', ['Variable ' SA_signal ' must be a vector.']);
      |         clear SA_signal;
      |         return;
      |     end
      | 
      |     SA_stime = str2num(get_param(gcb, 'stime'));
      |     if isempty(SA_stime) || SA_stime < -1 || (SA_stime < 0 && SA_stime > -1)
      |         set_param(gcb, 'stime', '-1');
      |         SA_stime = -1;
      |         warning('VAC:AttackController:After end', 'Sample time must be a positive double or -1 for inherited value.');
      |     end
      | 
      |     if SA_stime == 0 || SA_stime == -1
      |         SA_stime = evalin('base', 'Ts_base');
      |     end
      | 
      | 	SA_start = str2double(get_param(gcb, 'start'));
      | 	SA_start = SA_stime * ceil(SA_start/SA_stime);
      | 	signalstruct.time = SA_start:SA_stime:(SA_stime*(length(SA_signal) - 1) + SA_start);
      | 	signalstruct.signals.values = SA_signal;
      | 
      | 	if strcmp(get_param(gcb, 'afterend'), 'Cyclic repetition')
      | 		SA_end = str2double(get_param(gcr, 'StopTime'));
      | 		while signalstruct.time(end) < SA_end
      | 			signalstruct.signals.values = [signalstruct.signals.values signalstruct.signals.values];
      | 			signalstruct.time = [signalstruct.time signalstruct.time+(signalstruct.time(end)-signalstruct.time(1))];
      | 		end
      |     end
      | 
      |     signalstruct.time = signalstruct.time(:);
      | 	signalstruct.signals.values = signalstruct.signals.values(:);
      |     %assignin('base', 'signalstruct', signalstruct)
      |     set_param([gcb '/SignalIn'], 'VariableName', 'signalstruct');
      | 
      | 	clear SA_stime;
      | 	clear SA_start;
      | 	clear SA_signal;
      | 	clear SA_end;
      | end
      mask Display:
      | disp([get_param(gcb, 'switch_mode') '\n' get_param(gcb, 'atkMode')])
      | port_label('input', 1, 'signal in')
      | port_label('output', 1, 'signal out')
  xmeas5 attack controller : Subsystem  AncestorBlock=VAlib/Attack Controller  mask(Attack controller){switch_mode=Integrity attack, atkMode=No attack, start=1, duration=1, Value=0, signalin=[], stime=-1, afterend=Holding final value}
      mask prompts: switch_mode "Attack Type:"; atkMode "Attack Mode:"; Value "Integrity Attack Value:"; signalin "Signal variable:"; stime "Sample time:"; afterend "Output after final:"
      mask help:
      | Attack controller block controls an attack on choosen variable on the specified time.
      | Attack types: DoS, Integrity and custom signal attack.
      | Modes: Step attack on specified time, Interval to specified time, Periodic and no attack.
      mask TypeOptions switch_mode: Integrity attack | DOS attack | Custom attack
      mask Callback switch_mode:
      | SM_MaskEnables = get_param(gcb, 'MaskEnables');
      | switch get_param(gcb, 'switch_mode')
      |     case 'Integrity attack'
      |         set_param([gcb,'/Switch value'], 'Value', '1');
      |         SM_MaskEnables{5} = 'on';
      |         SM_MaskEnables{6} = 'off';
      |         SM_MaskEnables{7} = 'off';
      |         SM_MaskEnables{8} = 'off';
      |     case 'DOS attack'
      |         set_param([gcb,'/Switch value'], 'Value', '3');
      |         SM_MaskEnables{5} = 'off';
      |         SM_MaskEnables{6} = 'off';
      |         SM_MaskEnables{7} = 'off';
      |         SM_MaskEnables{8} = 'off';
      |     case 'Custom attack'
      |         set_param([gcb,'/Switch value'], 'Value', '2');
      |         SM_MaskEnables{5} = 'off';
      |         SM_MaskEnables{6} = 'on';
      |         SM_MaskEnables{7} = 'on';
      |         SM_MaskEnables{8} = 'on';
      | end
      | set_param(gcb,'MaskEnables',SM_MaskEnables);
      | clear SM_MaskEnables;
      | 
      | % creat or remove block for custom attack
      | if strcmpi(get_param(gcb, 'switch_mode'), 'Custom attack') && ~exists_block([gcb '/SignalIn']) % creat block
      |     if exists_block([gcb, '/ReplaceBlock']);
      |         delete_line(gcb, 'ReplaceBlock/1', 'Multiport Switch/3');
      |         delete_block([gcb '/ReplaceBlock']);
      |     end
      | 
      |     add_block('built-in/FromWorkspace', [gcb '/SignalIn'], 'Position', [50 400 120 430]);
      |     add_line(gcb, 'SignalIn/1', 'Multiport Switch/3', 'autorouting', 'on');
      |     %set params
      |     set_param([gcb '/SignalIn'], 'SampleTime', '0');
      |     %set_param([gcb '/SignalIn'], 'VariableName', '[]');
      |     set_param([gcb '/SignalIn'], 'Interpolate', 'on');
      |     set_param([gcb '/SignalIn'], 'ZeroCross', 'off');
      |     %set_param([gcb '/' name], 'OutputAfterFinalValue', 'Setting to zero');
      |     %set_param([gcb '/' name], 'OutputAfterFinalValue', 'Cyclic repetition');
      |     %set_param([gcb '/' name], 'OutputAfterFinalValue', 'Extrapolation');
      |     %set_param([gcb '/' name], 'OutputAfterFinalValue', 'Holding final value');
      | 
      |     % forward signal parameters if set
      |     SW_signal = get_param(gcb, 'signalin');
      |     if strcmp(SW_signal, '[]') || strcmp(SW_signal, '') % signal not set
      |         set_param(gcb, 'signalin', '[]');
      |         set_param([gcb '/SignalIn'], 'VariableName', '[]');
      |         clear SW_signal;
      |         return;
      |     else    % signal set
      |         % check signal
      |         if ~exist(SW_signal)
      |             set_param(gcb, 'signalin', '[]');
      |             set_param([gcb '/SignalIn'], 'VariableName', '[]');
      |             warning(['Variable ' SW_signal ' not found.']);
      |             clear SW_signal;
      |             return;
      |         end
      |         SW_signal = evalin('base', SW_signal);
      |         if ~isvector(SW_signal)
      |             set_param(gcb, 'signalin', '');
      |             set_param([gcb '/SignalIn'], 'VariableName', '[]');
      |             warning(['Variable ' SW_signal ' must be a vector.']);
      |             clear SW_signal;
      |             return;
      |         end
      |         SW_stime = str2num(get_param(gcb, 'stime'));
      |         if isempty(SW_stime) || SW_stime < -1 || (SW_stime < 0 && SW_stime > -1)
      |             set_param(gcb, 'stime', '-1');
      |             SW_stime = -1;
      |             warning('Sample time must be a positive double or -1 for inherited value.');
      |         end
      | 
      |         if SW_stime == 0 || SW_stime == -1
      |             SW_stime = evalin('base', 'Ts_base');
      |         end
      | 
      |         SW_start = str2num(get_param(gcb, 'start'));
      |         SW_start = SW_stime * ceil(SW_start/SW_stime);
      |         signalstruct.time = SW_start:SW_stime:(SW_stime*(length(SW_signal) - 1) + SW_start);
      |         signalstruct.signals.values = SW_signal;
      | 
      | 		if strcmp(get_param(gcb, 'afterend'), 'Cyclic repetition')
      | 			SW_end = str2double(get_param(gcr, 'StopTime'));
      | 			while signalstruct.time(end) < SW_end
      | 				signalstruct.signals.values = [signalstruct.signals.values signalstruct.signals.values];
      | 				signalstruct.time = [signalstruct.time signalstruct.time+(signalstruct.time(end)-signalstruct.time(1))];
      | 			end
      | 		end
      | 
      | 		signalstruct.signals.values = signalstruct.signals.values(:);
      | 		signalstruct.time = signalstruct.time(:);
      |         %assignin('base', 'signalstruct', signalstruct)
      |         set_param([gcb '/SignalIn'], 'VariableName', 'signalstruct');
      |     end
      | 
      |     clear SW_signal;
      | 	clear SW_start;
      |     clear SW_stime;
      | 	clear SW_end;
      | elseif ~strcmpi(get_param(gcb, 'switch_mode'), 'Custom attack') && exists_block([gcb '/SignalIn']) % delete block
      |     delete_line(gcb, 'SignalIn/1', 'Multiport Switch/3');
      |     delete_block([gcb '/SignalIn']);
      |     % replace with constant value
      |     add_block(['built-in/Constant'], [gcb '/ReplaceBlock'], 'Position', [50 400 120 430]);
      |     add_line(gcb, ['ReplaceBlock/1'], 'Multiport Switch/3', 'autorouting', 'on');
      | end
      mask TypeOptions atkMode: Attack Type Controller/atkMode
      mask Callback atkMode:
      | AM_MaskEnables = get_param(gcb, 'MaskEnables');
      | switch get_param(gcb, 'atkMode');
      |     case 'No attack'
      |         AM_MaskEnables{3} = 'off';
      |         AM_MaskEnables{4} = 'off';
      |     case 'Step attack'
      |         AM_MaskEnables{3} = 'on';
      |         AM_MaskEnables{4} = 'off';
      |     otherwise
      |         AM_MaskEnables{3} = 'on';
      |         AM_MaskEnables{4} = 'on';
      | end
      | set_param(gcb, 'MaskEnables', AM_MaskEnables);
      | 
      | clear AM_MaskEnables;
      mask Callback start:
      | SS_start = get_param(gcb, 'start');
      | if strcmp(SS_start, '') % empty
      |     set_param(gcb, 'start', '0');
      |     SS_start = 0;
      | end
      | SS_start = str2num(SS_start);
      | if isempty(SS_start)
      |     set_param(gcb, 'start', '0');
      |     SS_start = 0;
      |     warning('Parameter value must be a nimeric value.');
      | end
      | 
      | % set to the subsystem
      | set_param([gcb '/Attack Type Controller'], 'start', get_param(gcb, 'start'));
      | 
      | % get correct signal parameters
      | if strcmpi(get_param(gcb, 'switch_mode'),'custom attack')
      |     if ~exists_block([gcb '/SignalIn'])
      |         clear SS_start;
      |         return
      |     end
      |     % forward signal parameters if set
      |     SS_signal = get_param(gcb, 'signalin');
      |     if strcmp(SS_signal, '[]') || strcmp(SS_signal, '') % signal not set
      |         clear SS_signal;
      |         clear SS_start;
      |         return;
      |     else    % signal set
      |         SS_signal = evalin('base', SS_signal);
      |         SS_stime = str2num(get_param(gcb, 'stime'));
      |         if isempty(SS_stime) || SS_stime < -1 || (SS_stime < 0 && SS_stime > -1)
      |             clear SS_signal;
      |             clear SS_start;
      |             set_param(gcb, 'stime', '-1');
      |             SS_stime = -1;
      |             warning('Sample time must be a positve double or -1 for inherited value.')
      |         end
      | 
      |         if SS_stime == 0 || SS_stime == -1
      |             SS_stime = evalin('base', 'Ts_base');
      |         end
      | 
      | 
      |         signalstruct.time = SS_start:SS_stime:(SS_stime*(length(SS_signal) - 1) + SS_start);
      |         signalstruct.signals.values = SS_signal;
      | 
      | 		if strcmp(get_param(gcb, 'afterend'), 'Cyclic repetition')
      | 			SS_end = str2double(get_param(gcr, 'StopTime'));
      | 			while signalstruct.time(end) < SS_end
      | 				signalstruct.signals.values = [signalstruct.signals.values signalstruct.signals.values];
      | 				signalstruct.time = [signalstruct.time signalstruct.time+(signalstruct.time(end)-signalstruct.time(1))];
      | 			end
      | 		end
      | 
      | 		signalstruct.signals.values = signalstruct.signals.values(:);
      | 		signalstruct.time = signalstruct.time(:);
      |         %assignin('base', 'signalstruct', signalstruct)
      |         set_param([gcb '/SignalIn'], 'VariableName', 'signalstruct');
      | 		clear SS_signal;
      | 		clear SS_start;
      | 		clear SS_stime;
      | 		clear SS_end;
      |     end
      | 
      | end
      mask TypeOptions duration: Attack Type Controller/duration
      mask TypeOptions Value: Integrity attack value/Value
      mask Callback signalin:
      | if ~exists_block([gcb '/SignalIn'])
      |     return;
      | end
      | 
      | % forward signal parameters if set
      | SI_signal = get_param(gcb, 'signalin');
      | if strcmp(SI_signal, '[]') || strcmp(SI_signal, '') % signal not set
      |     set_param([gcb '/SignalIn'], 'VariableName', '[]');
      |     set_param(gcb, 'signalin', '[]');
      |     clear SI_signal;
      | else
      |     if ~exist(SI_signal)
      |         set_param(gcb, 'signalin', '[]');
      |         set_param([gcb '/SignalIn'], 'VariableName', '[]');
      |         warning('VAC:AttackController:Signal variable', ['Variable ' SI_signal ' not found.']);
      |         clear SI_signal;
      |         return;
      |     end
      | 
      |     SI_signal = evalin('base', SI_signal);
      |     if ~isvector(SI_signal)
      |         set_param(gcb, 'signalin', '[]');
      |         set_param([gcb '/SignalIn'], 'VariableName', '[]');
      |         warning('VAC:AttackController:Signal variable', ['Variable ' SI_signal ' must be a vector.']);
      |         clear SI_signal;
      |         return;
      |     end
      | 
      |     SI_stime = str2num(get_param(gcb, 'stime'));
      |     if isempty(SI_stime) || SI_stime < -1 || (SI_stime < 0 && SI_stime > -1)
      |         set_param(gcb, 'stime', '-1');
      |         SI_stime = -1;
      |         warning('VAC:AttackController:Signal variable', 'Sample time must be a positive double or -1 for inherited value.');
      |     end
      | 
      |     if SI_stime == 0 || SI_stime == -1
      |         SI_stime = evalin('base', 'Ts_base');
      |     end
      | 
      | 	SI_start = str2double(get_param(gcb, 'start'));
      | 	SI_start = SI_stime * ceil(SI_start/SI_stime);
      | 	signalstruct.time = SI_start:SI_stime:(SI_stime*(length(SI_signal) - 1) + SI_start);
      | 	signalstruct.signals.values = SI_signal;
      | 
      |     if strcmp(get_param(gcb, 'afterend'), 'Cyclic repetition')
      | 		SI_end = str2double(get_param(gcr, 'StopTime'));
      | 		while signalstruct.time(end) < SI_end
      | 			signalstruct.signals.values = [signalstruct.signals.values signalstruct.signals.values];
      | 			signalstruct.time = [signalstruct.time signalstruct.time+(signalstruct.time(end)-signalstruct.time(1))];
      | 		end
      | 	end
      | 
      | 	signalstruct.signals.values = signalstruct.signals.values(:);
      | 	signalstruct.time = signalstruct.time(:);
      |     %assignin('base', 'signalstruct', signalstruct)
      |     set_param([gcb '/SignalIn'], 'VariableName', 'signalstruct');
      | 	clear SI_stime;
      | 	clear SI_start;
      | 	clear SI_signal;
      | 	clear SI_end;
      | end
      mask Callback stime:
      | SQ_stime = get_param(gcb, 'stime');
      | if strcmp(SQ_stime, '') % empty
      |     set_param(gcb, 'stime', '-1');
      |     SQ_stime = -1;
      | end
      | SQ_stime = str2num(SQ_stime);
      | if isempty(SQ_stime)
      |     set_param(gcb, 'stime', '-1');
      |     SQ_stime = -1;
      |     warning('VAC:AttackController:Sample time','Sample time must be a positve double or -1 for inherited value.')
      | end
      | 
      | % get correct signal parameters
      | if strcmpi(get_param(gcb, 'switch_mode'),'custom attack')
      |     if ~exists_block([gcb '/SignalIn'])
      |         clear SS_start;
      |         return
      |     end
      |     % forward signal parameters if set
      |     SQ_signal = get_param(gcb, 'signalin');
      |     if strcmp(SQ_signal, '[]') || strcmp(SQ_signal, '') % signal not set
      |         clear SQ_signal;
      |         clear SQ_stime;
      |         return;
      |     else    % signal set
      |         SQ_signal = evalin('base', SQ_signal);
      |         if SQ_stime == 0 || SQ_stime == -1
      |             SQ_stime = evalin('base', 'Ts_base');
      |         end
      | 
      | 		SQ_start = str2double(get_param(gcb, 'start'));
      | 		SQ_start = SQ_stime * ceil(SQ_start/SQ_stime);
      | 		signalstruct.time = SQ_start:SQ_stime:(SQ_stime*(length(SQ_signal) - 1) + SQ_start);
      |         signalstruct.signals.values = SQ_signal;
      | 
      | 		if strcmp(get_param(gcb, 'afterend'), 'Cyclic repetition')
      | 			SQ_end = str2double(get_param(gcr, 'StopTime'));
      | 			while signalstruct.time(end) < SQ_end
      | 				signalstruct.signals.values = [signalstruct.signals.values signalstruct.signals.values];
      | 				signalstruct.time = [signalstruct.time signalstruct.time+(signalstruct.time(end)-signalstruct.time(1))];
      | 			end
      | 		end
      | 
      | 		signalstruct.signals.values = signalstruct.signals.values(:);
      | 		signalstruct.time = signalstruct.time(:);
      |         %assignin('base', 'signalstruct', signalstruct)
      |         set_param([gcb '/SignalIn'], 'VariableName', 'signalstruct');
      |     end
      | 	clear SQ_signal;
      | 	clear SQ_start;
      | 	clear SQ_stime;
      | 	clear SQ_end;
      | end
      mask TypeOptions afterend: Extrapolation | Setting to zero | Holding final value | Cyclic repetition
      mask Callback afterend:
      | if ~exists_block([gcb '/SignalIn'])
      |     return
      | end
      | 
      | % forward choosen value
      | if ~strcmp(get_param(gcb, 'afterend'), 'Cyclic repetition')
      | 	set_param([gcb '/SignalIn'], 'OutputAfterFinalValue', get_param(gcb, 'afterend'));
      | end
      | 
      | % forward signal parameters if set
      | SA_signal = get_param(gcb, 'signalin');
      | if strcmp(SA_signal, '[]') || strcmp(SA_signal, '') % signal not set
      |     set_param([gcb '/SignalIn'], 'VariableName', '[]');
      |     set_param(gcb, 'signalin', '[]');
      |     clear SA_signal;
      | else
      |     if ~exist(SA_signal)
      |         set_param(gcb, 'signalin', '[]');
      |         set_param([gcb '/SignalIn'], 'VariableName', '[]');
      |         warning('VAC:AttackController:After end', ['Variable ' SA_signal ' not found.']);
      |         clear SA_signal;
      |         return;
      |     end
      | 
      |     SA_signal = evalin('base', SA_signal);
      |     if ~isvector(SA_signal)
      |         set_param(gcb, 'signalin', '[]');
      |         set_param([gcb '/SignalIn'], 'VariableName', '[]');
      |         warning('VAC:AttackController:After end', ['Variable ' SA_signal ' must be a vector.']);
      |         clear SA_signal;
      |         return;
      |     end
      | 
      |     SA_stime = str2num(get_param(gcb, 'stime'));
      |     if isempty(SA_stime) || SA_stime < -1 || (SA_stime < 0 && SA_stime > -1)
      |         set_param(gcb, 'stime', '-1');
      |         SA_stime = -1;
      |         warning('VAC:AttackController:After end', 'Sample time must be a positive double or -1 for inherited value.');
      |     end
      | 
      |     if SA_stime == 0 || SA_stime == -1
      |         SA_stime = evalin('base', 'Ts_base');
      |     end
      | 
      | 	SA_start = str2double(get_param(gcb, 'start'));
      | 	SA_start = SA_stime * ceil(SA_start/SA_stime);
      | 	signalstruct.time = SA_start:SA_stime:(SA_stime*(length(SA_signal) - 1) + SA_start);
      | 	signalstruct.signals.values = SA_signal;
      | 
      | 	if strcmp(get_param(gcb, 'afterend'), 'Cyclic repetition')
      | 		SA_end = str2double(get_param(gcr, 'StopTime'));
      | 		while signalstruct.time(end) < SA_end
      | 			signalstruct.signals.values = [signalstruct.signals.values signalstruct.signals.values];
      | 			signalstruct.time = [signalstruct.time signalstruct.time+(signalstruct.time(end)-signalstruct.time(1))];
      | 		end
      |     end
      | 
      |     signalstruct.time = signalstruct.time(:);
      | 	signalstruct.signals.values = signalstruct.signals.values(:);
      |     %assignin('base', 'signalstruct', signalstruct)
      |     set_param([gcb '/SignalIn'], 'VariableName', 'signalstruct');
      | 
      | 	clear SA_stime;
      | 	clear SA_start;
      | 	clear SA_signal;
      | 	clear SA_end;
      | end
      mask Display:
      | disp([get_param(gcb, 'switch_mode') '\n' get_param(gcb, 'atkMode')])
      | port_label('input', 1, 'signal in')
      | port_label('output', 1, 'signal out')
  xmeas6 attack controller : Subsystem  AncestorBlock=VAlib/Attack Controller  mask(Attack controller){switch_mode=Integrity attack, atkMode=No attack, start=1, duration=1, Value=0, signalin=[], stime=-1, afterend=Holding final value}
